simulink model "IEEE118_FULL_seed17_GFOL_RL_percgfor091_PyStable"  (R2023a)
(part 1 of 3)
settings: Solver=ode1  StartTime=0.0  StopTime=sim_config.Tsim  RelTol=1e-3
undefined symbols (not defined in the file): sim_config
libraries: myLibrary x561, spsThreePhaseVIMeasurementLib x250, spsPower3phInstantaneousLib x137, spspowerguiLib x1
settings Model: Creator=Francesca  LastModifiedBy=Francesca

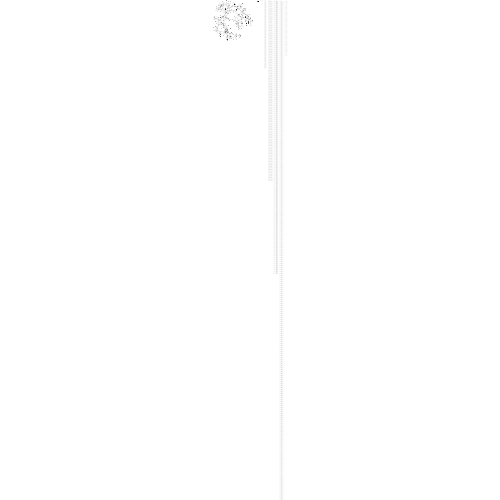
[thumbnail: Simulink's stored preview of the top-level diagram]
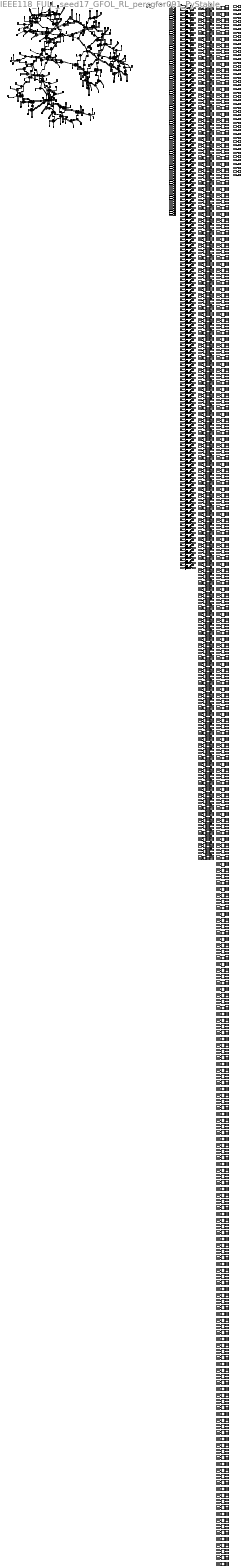
== system IEEE118_FULL_seed17_GFOL_RL_percgfor091_PyStable ==
  note: Line-to-Line Voltages
  note: Line-to-Neutral Voltages
  note: Power Measurements
  note: qd0 transforms
  note: omega
  BUS-1 : spsThreePhaseVIMeasurementLib/Three-Phase V-I Measurement  VoltageMeasurement=phase-to-phase  SetLabelV=on  LabelV=V_ll_1  Vpu=off  VpuLL=off  CurrentMeasurement=yes  SetLabelI=on  LabelI=I_1  Ipu=off  Pbase=100e6  Vbase=500e3  OutputType=Complex  PhasorSimulation=off  PSBequivalent=0
  BUS-100 : spsThreePhaseVIMeasurementLib/Three-Phase V-I Measurement  VoltageMeasurement=phase-to-phase  SetLabelV=on  LabelV=V_ll_100  Vpu=off  VpuLL=off  CurrentMeasurement=yes  SetLabelI=on  LabelI=I_100  Ipu=off  Pbase=100e6  Vbase=500e3  OutputType=Complex  PhasorSimulation=off  PSBequivalent=0
  BUS-101 : spsThreePhaseVIMeasurementLib/Three-Phase V-I Measurement  VoltageMeasurement=phase-to-phase  SetLabelV=on  LabelV=V_ll_101  Vpu=off  VpuLL=off  CurrentMeasurement=yes  SetLabelI=on  LabelI=I_101  Ipu=off  Pbase=100e6  Vbase=500e3  OutputType=Complex  PhasorSimulation=off  PSBequivalent=0
  BUS-102 : spsThreePhaseVIMeasurementLib/Three-Phase V-I Measurement  VoltageMeasurement=phase-to-phase  SetLabelV=on  LabelV=V_ll_102  Vpu=off  VpuLL=off  CurrentMeasurement=yes  SetLabelI=on  LabelI=I_102  Ipu=off  Pbase=100e6  Vbase=500e3  OutputType=Complex  PhasorSimulation=off  PSBequivalent=0
  BUS-103 : spsThreePhaseVIMeasurementLib/Three-Phase V-I Measurement  VoltageMeasurement=phase-to-phase  SetLabelV=on  LabelV=V_ll_103  Vpu=off  VpuLL=off  CurrentMeasurement=yes  SetLabelI=on  LabelI=I_103  Ipu=off  Pbase=100e6  Vbase=500e3  OutputType=Complex  PhasorSimulation=off  PSBequivalent=0
  BUS-104 : spsThreePhaseVIMeasurementLib/Three-Phase V-I Measurement  VoltageMeasurement=phase-to-phase  SetLabelV=on  LabelV=V_ll_104  Vpu=off  VpuLL=off  CurrentMeasurement=yes  SetLabelI=on  LabelI=I_104  Ipu=off  Pbase=100e6  Vbase=500e3  OutputType=Complex  PhasorSimulation=off  PSBequivalent=0
  BUS-105 : spsThreePhaseVIMeasurementLib/Three-Phase V-I Measurement  VoltageMeasurement=phase-to-phase  SetLabelV=on  LabelV=V_ll_105  Vpu=off  VpuLL=off  CurrentMeasurement=yes  SetLabelI=on  LabelI=I_105  Ipu=off  Pbase=100e6  Vbase=500e3  OutputType=Complex  PhasorSimulation=off  PSBequivalent=0
  BUS-106 : spsThreePhaseVIMeasurementLib/Three-Phase V-I Measurement  VoltageMeasurement=phase-to-phase  SetLabelV=on  LabelV=V_ll_106  Vpu=off  VpuLL=off  CurrentMeasurement=yes  SetLabelI=on  LabelI=I_106  Ipu=off  Pbase=100e6  Vbase=500e3  OutputType=Complex  PhasorSimulation=off  PSBequivalent=0
  BUS-107 : spsThreePhaseVIMeasurementLib/Three-Phase V-I Measurement  VoltageMeasurement=phase-to-phase  SetLabelV=on  LabelV=V_ll_107  Vpu=off  VpuLL=off  CurrentMeasurement=yes  SetLabelI=on  LabelI=I_107  Ipu=off  Pbase=100e6  Vbase=500e3  OutputType=Complex  PhasorSimulation=off  PSBequivalent=0
  BUS-108 : spsThreePhaseVIMeasurementLib/Three-Phase V-I Measurement  VoltageMeasurement=phase-to-phase  SetLabelV=on  LabelV=V_ll_108  Vpu=off  VpuLL=off  CurrentMeasurement=yes  SetLabelI=on  LabelI=I_108  Ipu=off  Pbase=100e6  Vbase=500e3  OutputType=Complex  PhasorSimulation=off  PSBequivalent=0
  BUS-109 : spsThreePhaseVIMeasurementLib/Three-Phase V-I Measurement  VoltageMeasurement=phase-to-phase  SetLabelV=on  LabelV=V_ll_109  Vpu=off  VpuLL=off  CurrentMeasurement=yes  SetLabelI=on  LabelI=I_109  Ipu=off  Pbase=100e6  Vbase=500e3  OutputType=Complex  PhasorSimulation=off  PSBequivalent=0
  BUS-11 : spsThreePhaseVIMeasurementLib/Three-Phase V-I Measurement  VoltageMeasurement=phase-to-phase  SetLabelV=on  LabelV=V_ll_11  Vpu=off  VpuLL=off  CurrentMeasurement=yes  SetLabelI=on  LabelI=I_11  Ipu=off  Pbase=100e6  Vbase=500e3  OutputType=Complex  PhasorSimulation=off  PSBequivalent=0
  BUS-110 : spsThreePhaseVIMeasurementLib/Three-Phase V-I Measurement  VoltageMeasurement=phase-to-phase  SetLabelV=on  LabelV=V_ll_110  Vpu=off  VpuLL=off  CurrentMeasurement=yes  SetLabelI=on  LabelI=I_110  Ipu=off  Pbase=100e6  Vbase=500e3  OutputType=Complex  PhasorSimulation=off  PSBequivalent=0
  BUS-112 : spsThreePhaseVIMeasurementLib/Three-Phase V-I Measurement  VoltageMeasurement=phase-to-phase  SetLabelV=on  LabelV=V_ll_112  Vpu=off  VpuLL=off  CurrentMeasurement=yes  SetLabelI=on  LabelI=I_112  Ipu=off  Pbase=100e6  Vbase=500e3  OutputType=Complex  PhasorSimulation=off  PSBequivalent=0
  BUS-113 : spsThreePhaseVIMeasurementLib/Three-Phase V-I Measurement  VoltageMeasurement=phase-to-phase  SetLabelV=on  LabelV=V_ll_113  Vpu=off  VpuLL=off  CurrentMeasurement=yes  SetLabelI=on  LabelI=I_113  Ipu=off  Pbase=100e6  Vbase=500e3  OutputType=Complex  PhasorSimulation=off  PSBequivalent=0
  BUS-114 : spsThreePhaseVIMeasurementLib/Three-Phase V-I Measurement  VoltageMeasurement=phase-to-phase  SetLabelV=on  LabelV=V_ll_114  Vpu=off  VpuLL=off  CurrentMeasurement=yes  SetLabelI=on  LabelI=I_114  Ipu=off  Pbase=100e6  Vbase=500e3  OutputType=Complex  PhasorSimulation=off  PSBequivalent=0
  BUS-115 : spsThreePhaseVIMeasurementLib/Three-Phase V-I Measurement  VoltageMeasurement=phase-to-phase  SetLabelV=on  LabelV=V_ll_115  Vpu=off  VpuLL=off  CurrentMeasurement=yes  SetLabelI=on  LabelI=I_115  Ipu=off  Pbase=100e6  Vbase=500e3  OutputType=Complex  PhasorSimulation=off  PSBequivalent=0
  BUS-117 : spsThreePhaseVIMeasurementLib/Three-Phase V-I Measurement  VoltageMeasurement=phase-to-phase  SetLabelV=on  LabelV=V_ll_117  Vpu=off  VpuLL=off  CurrentMeasurement=yes  SetLabelI=on  LabelI=I_117  Ipu=off  Pbase=100e6  Vbase=500e3  OutputType=Complex  PhasorSimulation=off  PSBequivalent=0
  BUS-118 : spsThreePhaseVIMeasurementLib/Three-Phase V-I Measurement  VoltageMeasurement=phase-to-phase  SetLabelV=on  LabelV=V_ll_118  Vpu=off  VpuLL=off  CurrentMeasurement=yes  SetLabelI=on  LabelI=I_118  Ipu=off  Pbase=100e6  Vbase=500e3  OutputType=Complex  PhasorSimulation=off  PSBequivalent=0
  BUS-12 : spsThreePhaseVIMeasurementLib/Three-Phase V-I Measurement  VoltageMeasurement=phase-to-phase  SetLabelV=on  LabelV=V_ll_12  Vpu=off  VpuLL=off  CurrentMeasurement=yes  SetLabelI=on  LabelI=I_12  Ipu=off  Pbase=100e6  Vbase=500e3  OutputType=Complex  PhasorSimulation=off  PSBequivalent=0
  BUS-13 : spsThreePhaseVIMeasurementLib/Three-Phase V-I Measurement  VoltageMeasurement=phase-to-phase  SetLabelV=on  LabelV=V_ll_13  Vpu=off  VpuLL=off  CurrentMeasurement=yes  SetLabelI=on  LabelI=I_13  Ipu=off  Pbase=100e6  Vbase=500e3  OutputType=Complex  PhasorSimulation=off  PSBequivalent=0
  BUS-14 : spsThreePhaseVIMeasurementLib/Three-Phase V-I Measurement  VoltageMeasurement=phase-to-phase  SetLabelV=on  LabelV=V_ll_14  Vpu=off  VpuLL=off  CurrentMeasurement=yes  SetLabelI=on  LabelI=I_14  Ipu=off  Pbase=100e6  Vbase=500e3  OutputType=Complex  PhasorSimulation=off  PSBequivalent=0
  BUS-15 : spsThreePhaseVIMeasurementLib/Three-Phase V-I Measurement  VoltageMeasurement=phase-to-phase  SetLabelV=on  LabelV=V_ll_15  Vpu=off  VpuLL=off  CurrentMeasurement=yes  SetLabelI=on  LabelI=I_15  Ipu=off  Pbase=100e6  Vbase=500e3  OutputType=Complex  PhasorSimulation=off  PSBequivalent=0
  BUS-16 : spsThreePhaseVIMeasurementLib/Three-Phase V-I Measurement  VoltageMeasurement=phase-to-phase  SetLabelV=on  LabelV=V_ll_16  Vpu=off  VpuLL=off  CurrentMeasurement=yes  SetLabelI=on  LabelI=I_16  Ipu=off  Pbase=100e6  Vbase=500e3  OutputType=Complex  PhasorSimulation=off  PSBequivalent=0
  BUS-17 : spsThreePhaseVIMeasurementLib/Three-Phase V-I Measurement  VoltageMeasurement=phase-to-phase  SetLabelV=on  LabelV=V_ll_17  Vpu=off  VpuLL=off  CurrentMeasurement=yes  SetLabelI=on  LabelI=I_17  Ipu=off  Pbase=100e6  Vbase=500e3  OutputType=Complex  PhasorSimulation=off  PSBequivalent=0
  BUS-18 : spsThreePhaseVIMeasurementLib/Three-Phase V-I Measurement  VoltageMeasurement=phase-to-phase  SetLabelV=on  LabelV=V_ll_18  Vpu=off  VpuLL=off  CurrentMeasurement=yes  SetLabelI=on  LabelI=I_18  Ipu=off  Pbase=100e6  Vbase=500e3  OutputType=Complex  PhasorSimulation=off  PSBequivalent=0
  BUS-19 : spsThreePhaseVIMeasurementLib/Three-Phase V-I Measurement  VoltageMeasurement=phase-to-phase  SetLabelV=on  LabelV=V_ll_19  Vpu=off  VpuLL=off  CurrentMeasurement=yes  SetLabelI=on  LabelI=I_19  Ipu=off  Pbase=100e6  Vbase=500e3  OutputType=Complex  PhasorSimulation=off  PSBequivalent=0
  BUS-2 : spsThreePhaseVIMeasurementLib/Three-Phase V-I Measurement  VoltageMeasurement=phase-to-phase  SetLabelV=on  LabelV=V_ll_2  Vpu=off  VpuLL=off  CurrentMeasurement=yes  SetLabelI=on  LabelI=I_2  Ipu=off  Pbase=100e6  Vbase=500e3  OutputType=Complex  PhasorSimulation=off  PSBequivalent=0
  BUS-20 : spsThreePhaseVIMeasurementLib/Three-Phase V-I Measurement  VoltageMeasurement=phase-to-phase  SetLabelV=on  LabelV=V_ll_20  Vpu=off  VpuLL=off  CurrentMeasurement=yes  SetLabelI=on  LabelI=I_20  Ipu=off  Pbase=100e6  Vbase=500e3  OutputType=Complex  PhasorSimulation=off  PSBequivalent=0
  BUS-21 : spsThreePhaseVIMeasurementLib/Three-Phase V-I Measurement  VoltageMeasurement=phase-to-phase  SetLabelV=on  LabelV=V_ll_21  Vpu=off  VpuLL=off  CurrentMeasurement=yes  SetLabelI=on  LabelI=I_21  Ipu=off  Pbase=100e6  Vbase=500e3  OutputType=Complex  PhasorSimulation=off  PSBequivalent=0
  BUS-22 : spsThreePhaseVIMeasurementLib/Three-Phase V-I Measurement  VoltageMeasurement=phase-to-phase  SetLabelV=on  LabelV=V_ll_22  Vpu=off  VpuLL=off  CurrentMeasurement=yes  SetLabelI=on  LabelI=I_22  Ipu=off  Pbase=100e6  Vbase=500e3  OutputType=Complex  PhasorSimulation=off  PSBequivalent=0
  BUS-23 : spsThreePhaseVIMeasurementLib/Three-Phase V-I Measurement  VoltageMeasurement=phase-to-phase  SetLabelV=on  LabelV=V_ll_23  Vpu=off  VpuLL=off  CurrentMeasurement=yes  SetLabelI=on  LabelI=I_23  Ipu=off  Pbase=100e6  Vbase=500e3  OutputType=Complex  PhasorSimulation=off  PSBequivalent=0
  BUS-24 : spsThreePhaseVIMeasurementLib/Three-Phase V-I Measurement  VoltageMeasurement=phase-to-phase  SetLabelV=on  LabelV=V_ll_24  Vpu=off  VpuLL=off  CurrentMeasurement=yes  SetLabelI=on  LabelI=I_24  Ipu=off  Pbase=100e6  Vbase=500e3  OutputType=Complex  PhasorSimulation=off  PSBequivalent=0
  BUS-25 : spsThreePhaseVIMeasurementLib/Three-Phase V-I Measurement  VoltageMeasurement=phase-to-phase  SetLabelV=on  LabelV=V_ll_25  Vpu=off  VpuLL=off  CurrentMeasurement=yes  SetLabelI=on  LabelI=I_25  Ipu=off  Pbase=100e6  Vbase=500e3  OutputType=Complex  PhasorSimulation=off  PSBequivalent=0
  BUS-26 : spsThreePhaseVIMeasurementLib/Three-Phase V-I Measurement  VoltageMeasurement=phase-to-phase  SetLabelV=on  LabelV=V_ll_26  Vpu=off  VpuLL=off  CurrentMeasurement=yes  SetLabelI=on  LabelI=I_26  Ipu=off  Pbase=100e6  Vbase=500e3  OutputType=Complex  PhasorSimulation=off  PSBequivalent=0
  BUS-27 : spsThreePhaseVIMeasurementLib/Three-Phase V-I Measurement  VoltageMeasurement=phase-to-phase  SetLabelV=on  LabelV=V_ll_27  Vpu=off  VpuLL=off  CurrentMeasurement=yes  SetLabelI=on  LabelI=I_27  Ipu=off  Pbase=100e6  Vbase=500e3  OutputType=Complex  PhasorSimulation=off  PSBequivalent=0
  BUS-28 : spsThreePhaseVIMeasurementLib/Three-Phase V-I Measurement  VoltageMeasurement=phase-to-phase  SetLabelV=on  LabelV=V_ll_28  Vpu=off  VpuLL=off  CurrentMeasurement=yes  SetLabelI=on  LabelI=I_28  Ipu=off  Pbase=100e6  Vbase=500e3  OutputType=Complex  PhasorSimulation=off  PSBequivalent=0
  BUS-29 : spsThreePhaseVIMeasurementLib/Three-Phase V-I Measurement  VoltageMeasurement=phase-to-phase  SetLabelV=on  LabelV=V_ll_29  Vpu=off  VpuLL=off  CurrentMeasurement=yes  SetLabelI=on  LabelI=I_29  Ipu=off  Pbase=100e6  Vbase=500e3  OutputType=Complex  PhasorSimulation=off  PSBequivalent=0
  BUS-3 : spsThreePhaseVIMeasurementLib/Three-Phase V-I Measurement  VoltageMeasurement=phase-to-phase  SetLabelV=on  LabelV=V_ll_3  Vpu=off  VpuLL=off  CurrentMeasurement=yes  SetLabelI=on  LabelI=I_3  Ipu=off  Pbase=100e6  Vbase=500e3  OutputType=Complex  PhasorSimulation=off  PSBequivalent=0
  BUS-30 : spsThreePhaseVIMeasurementLib/Three-Phase V-I Measurement  VoltageMeasurement=phase-to-phase  SetLabelV=on  LabelV=V_ll_30  Vpu=off  VpuLL=off  CurrentMeasurement=yes  SetLabelI=on  LabelI=I_30  Ipu=off  Pbase=100e6  Vbase=500e3  OutputType=Complex  PhasorSimulation=off  PSBequivalent=0
  BUS-31 : spsThreePhaseVIMeasurementLib/Three-Phase V-I Measurement  VoltageMeasurement=phase-to-phase  SetLabelV=on  LabelV=V_ll_31  Vpu=off  VpuLL=off  CurrentMeasurement=yes  SetLabelI=on  LabelI=I_31  Ipu=off  Pbase=100e6  Vbase=500e3  OutputType=Complex  PhasorSimulation=off  PSBequivalent=0
  BUS-32 : spsThreePhaseVIMeasurementLib/Three-Phase V-I Measurement  VoltageMeasurement=phase-to-phase  SetLabelV=on  LabelV=V_ll_32  Vpu=off  VpuLL=off  CurrentMeasurement=yes  SetLabelI=on  LabelI=I_32  Ipu=off  Pbase=100e6  Vbase=500e3  OutputType=Complex  PhasorSimulation=off  PSBequivalent=0
  BUS-33 : spsThreePhaseVIMeasurementLib/Three-Phase V-I Measurement  VoltageMeasurement=phase-to-phase  SetLabelV=on  LabelV=V_ll_33  Vpu=off  VpuLL=off  CurrentMeasurement=yes  SetLabelI=on  LabelI=I_33  Ipu=off  Pbase=100e6  Vbase=500e3  OutputType=Complex  PhasorSimulation=off  PSBequivalent=0
  BUS-34 : spsThreePhaseVIMeasurementLib/Three-Phase V-I Measurement  VoltageMeasurement=phase-to-phase  SetLabelV=on  LabelV=V_ll_34  Vpu=off  VpuLL=off  CurrentMeasurement=yes  SetLabelI=on  LabelI=I_34  Ipu=off  Pbase=100e6  Vbase=500e3  OutputType=Complex  PhasorSimulation=off  PSBequivalent=0
  BUS-35 : spsThreePhaseVIMeasurementLib/Three-Phase V-I Measurement  VoltageMeasurement=phase-to-phase  SetLabelV=on  LabelV=V_ll_35  Vpu=off  VpuLL=off  CurrentMeasurement=yes  SetLabelI=on  LabelI=I_35  Ipu=off  Pbase=100e6  Vbase=500e3  OutputType=Complex  PhasorSimulation=off  PSBequivalent=0
  BUS-36 : spsThreePhaseVIMeasurementLib/Three-Phase V-I Measurement  VoltageMeasurement=phase-to-phase  SetLabelV=on  LabelV=V_ll_36  Vpu=off  VpuLL=off  CurrentMeasurement=yes  SetLabelI=on  LabelI=I_36  Ipu=off  Pbase=100e6  Vbase=500e3  OutputType=Complex  PhasorSimulation=off  PSBequivalent=0
  BUS-37 : spsThreePhaseVIMeasurementLib/Three-Phase V-I Measurement  VoltageMeasurement=phase-to-phase  SetLabelV=on  LabelV=V_ll_37  Vpu=off  VpuLL=off  CurrentMeasurement=yes  SetLabelI=on  LabelI=I_37  Ipu=off  Pbase=100e6  Vbase=500e3  OutputType=Complex  PhasorSimulation=off  PSBequivalent=0
  BUS-38 : spsThreePhaseVIMeasurementLib/Three-Phase V-I Measurement  VoltageMeasurement=phase-to-phase  SetLabelV=on  LabelV=V_ll_38  Vpu=off  VpuLL=off  CurrentMeasurement=yes  SetLabelI=on  LabelI=I_38  Ipu=off  Pbase=100e6  Vbase=500e3  OutputType=Complex  PhasorSimulation=off  PSBequivalent=0
  BUS-39 : spsThreePhaseVIMeasurementLib/Three-Phase V-I Measurement  VoltageMeasurement=phase-to-phase  SetLabelV=on  LabelV=V_ll_39  Vpu=off  VpuLL=off  CurrentMeasurement=yes  SetLabelI=on  LabelI=I_39  Ipu=off  Pbase=100e6  Vbase=500e3  OutputType=Complex  PhasorSimulation=off  PSBequivalent=0
  BUS-4 : spsThreePhaseVIMeasurementLib/Three-Phase V-I Measurement  VoltageMeasurement=phase-to-phase  SetLabelV=on  LabelV=V_ll_4  Vpu=off  VpuLL=off  CurrentMeasurement=yes  SetLabelI=on  LabelI=I_4  Ipu=off  Pbase=100e6  Vbase=500e3  OutputType=Complex  PhasorSimulation=off  PSBequivalent=0
  BUS-40 : spsThreePhaseVIMeasurementLib/Three-Phase V-I Measurement  VoltageMeasurement=phase-to-phase  SetLabelV=on  LabelV=V_ll_40  Vpu=off  VpuLL=off  CurrentMeasurement=yes  SetLabelI=on  LabelI=I_40  Ipu=off  Pbase=100e6  Vbase=500e3  OutputType=Complex  PhasorSimulation=off  PSBequivalent=0
  BUS-41 : spsThreePhaseVIMeasurementLib/Three-Phase V-I Measurement  VoltageMeasurement=phase-to-phase  SetLabelV=on  LabelV=V_ll_41  Vpu=off  VpuLL=off  CurrentMeasurement=yes  SetLabelI=on  LabelI=I_41  Ipu=off  Pbase=100e6  Vbase=500e3  OutputType=Complex  PhasorSimulation=off  PSBequivalent=0
  BUS-42 : spsThreePhaseVIMeasurementLib/Three-Phase V-I Measurement  VoltageMeasurement=phase-to-phase  SetLabelV=on  LabelV=V_ll_42  Vpu=off  VpuLL=off  CurrentMeasurement=yes  SetLabelI=on  LabelI=I_42  Ipu=off  Pbase=100e6  Vbase=500e3  OutputType=Complex  PhasorSimulation=off  PSBequivalent=0
  BUS-43 : spsThreePhaseVIMeasurementLib/Three-Phase V-I Measurement  VoltageMeasurement=phase-to-phase  SetLabelV=on  LabelV=V_ll_43  Vpu=off  VpuLL=off  CurrentMeasurement=yes  SetLabelI=on  LabelI=I_43  Ipu=off  Pbase=100e6  Vbase=500e3  OutputType=Complex  PhasorSimulation=off  PSBequivalent=0
  BUS-44 : spsThreePhaseVIMeasurementLib/Three-Phase V-I Measurement  VoltageMeasurement=phase-to-phase  SetLabelV=on  LabelV=V_ll_44  Vpu=off  VpuLL=off  CurrentMeasurement=yes  SetLabelI=on  LabelI=I_44  Ipu=off  Pbase=100e6  Vbase=500e3  OutputType=Complex  PhasorSimulation=off  PSBequivalent=0
  BUS-45 : spsThreePhaseVIMeasurementLib/Three-Phase V-I Measurement  VoltageMeasurement=phase-to-phase  SetLabelV=on  LabelV=V_ll_45  Vpu=off  VpuLL=off  CurrentMeasurement=yes  SetLabelI=on  LabelI=I_45  Ipu=off  Pbase=100e6  Vbase=500e3  OutputType=Complex  PhasorSimulation=off  PSBequivalent=0
  BUS-46 : spsThreePhaseVIMeasurementLib/Three-Phase V-I Measurement  VoltageMeasurement=phase-to-phase  SetLabelV=on  LabelV=V_ll_46  Vpu=off  VpuLL=off  CurrentMeasurement=yes  SetLabelI=on  LabelI=I_46  Ipu=off  Pbase=100e6  Vbase=500e3  OutputType=Complex  PhasorSimulation=off  PSBequivalent=0
  BUS-47 : spsThreePhaseVIMeasurementLib/Three-Phase V-I Measurement  VoltageMeasurement=phase-to-phase  SetLabelV=on  LabelV=V_ll_47  Vpu=off  VpuLL=off  CurrentMeasurement=yes  SetLabelI=on  LabelI=I_47  Ipu=off  Pbase=100e6  Vbase=500e3  OutputType=Complex  PhasorSimulation=off  PSBequivalent=0
  BUS-48 : spsThreePhaseVIMeasurementLib/Three-Phase V-I Measurement  VoltageMeasurement=phase-to-phase  SetLabelV=on  LabelV=V_ll_48  Vpu=off  VpuLL=off  CurrentMeasurement=yes  SetLabelI=on  LabelI=I_48  Ipu=off  Pbase=100e6  Vbase=500e3  OutputType=Complex  PhasorSimulation=off  PSBequivalent=0
  BUS-49 : spsThreePhaseVIMeasurementLib/Three-Phase V-I Measurement  VoltageMeasurement=phase-to-phase  SetLabelV=on  LabelV=V_ll_49  Vpu=off  VpuLL=off  CurrentMeasurement=yes  SetLabelI=on  LabelI=I_49  Ipu=off  Pbase=100e6  Vbase=500e3  OutputType=Complex  PhasorSimulation=off  PSBequivalent=0
  BUS-5 : spsThreePhaseVIMeasurementLib/Three-Phase V-I Measurement  VoltageMeasurement=phase-to-phase  SetLabelV=on  LabelV=V_ll_5  Vpu=off  VpuLL=off  CurrentMeasurement=yes  SetLabelI=on  LabelI=I_5  Ipu=off  Pbase=100e6  Vbase=500e3  OutputType=Complex  PhasorSimulation=off  PSBequivalent=0
  BUS-50 : spsThreePhaseVIMeasurementLib/Three-Phase V-I Measurement  VoltageMeasurement=phase-to-phase  SetLabelV=on  LabelV=V_ll_50  Vpu=off  VpuLL=off  CurrentMeasurement=yes  SetLabelI=on  LabelI=I_50  Ipu=off  Pbase=100e6  Vbase=500e3  OutputType=Complex  PhasorSimulation=off  PSBequivalent=0
  BUS-51 : spsThreePhaseVIMeasurementLib/Three-Phase V-I Measurement  VoltageMeasurement=phase-to-phase  SetLabelV=on  LabelV=V_ll_51  Vpu=off  VpuLL=off  CurrentMeasurement=yes  SetLabelI=on  LabelI=I_51  Ipu=off  Pbase=100e6  Vbase=500e3  OutputType=Complex  PhasorSimulation=off  PSBequivalent=0
  BUS-52 : spsThreePhaseVIMeasurementLib/Three-Phase V-I Measurement  VoltageMeasurement=phase-to-phase  SetLabelV=on  LabelV=V_ll_52  Vpu=off  VpuLL=off  CurrentMeasurement=yes  SetLabelI=on  LabelI=I_52  Ipu=off  Pbase=100e6  Vbase=500e3  OutputType=Complex  PhasorSimulation=off  PSBequivalent=0
  BUS-53 : spsThreePhaseVIMeasurementLib/Three-Phase V-I Measurement  VoltageMeasurement=phase-to-phase  SetLabelV=on  LabelV=V_ll_53  Vpu=off  VpuLL=off  CurrentMeasurement=yes  SetLabelI=on  LabelI=I_53  Ipu=off  Pbase=100e6  Vbase=500e3  OutputType=Complex  PhasorSimulation=off  PSBequivalent=0
  BUS-54 : spsThreePhaseVIMeasurementLib/Three-Phase V-I Measurement  VoltageMeasurement=phase-to-phase  SetLabelV=on  LabelV=V_ll_54  Vpu=off  VpuLL=off  CurrentMeasurement=yes  SetLabelI=on  LabelI=I_54  Ipu=off  Pbase=100e6  Vbase=500e3  OutputType=Complex  PhasorSimulation=off  PSBequivalent=0
  BUS-55 : spsThreePhaseVIMeasurementLib/Three-Phase V-I Measurement  VoltageMeasurement=phase-to-phase  SetLabelV=on  LabelV=V_ll_55  Vpu=off  VpuLL=off  CurrentMeasurement=yes  SetLabelI=on  LabelI=I_55  Ipu=off  Pbase=100e6  Vbase=500e3  OutputType=Complex  PhasorSimulation=off  PSBequivalent=0
  BUS-56 : spsThreePhaseVIMeasurementLib/Three-Phase V-I Measurement  VoltageMeasurement=phase-to-phase  SetLabelV=on  LabelV=V_ll_56  Vpu=off  VpuLL=off  CurrentMeasurement=yes  SetLabelI=on  LabelI=I_56  Ipu=off  Pbase=100e6  Vbase=500e3  OutputType=Complex  PhasorSimulation=off  PSBequivalent=0
  BUS-57 : spsThreePhaseVIMeasurementLib/Three-Phase V-I Measurement  VoltageMeasurement=phase-to-phase  SetLabelV=on  LabelV=V_ll_57  Vpu=off  VpuLL=off  CurrentMeasurement=yes  SetLabelI=on  LabelI=I_57  Ipu=off  Pbase=100e6  Vbase=500e3  OutputType=Complex  PhasorSimulation=off  PSBequivalent=0
  BUS-58 : spsThreePhaseVIMeasurementLib/Three-Phase V-I Measurement  VoltageMeasurement=phase-to-phase  SetLabelV=on  LabelV=V_ll_58  Vpu=off  VpuLL=off  CurrentMeasurement=yes  SetLabelI=on  LabelI=I_58  Ipu=off  Pbase=100e6  Vbase=500e3  OutputType=Complex  PhasorSimulation=off  PSBequivalent=0
  BUS-59 : spsThreePhaseVIMeasurementLib/Three-Phase V-I Measurement  VoltageMeasurement=phase-to-phase  SetLabelV=on  LabelV=V_ll_59  Vpu=off  VpuLL=off  CurrentMeasurement=yes  SetLabelI=on  LabelI=I_59  Ipu=off  Pbase=100e6  Vbase=500e3  OutputType=Complex  PhasorSimulation=off  PSBequivalent=0
  BUS-6 : spsThreePhaseVIMeasurementLib/Three-Phase V-I Measurement  VoltageMeasurement=phase-to-phase  SetLabelV=on  LabelV=V_ll_6  Vpu=off  VpuLL=off  CurrentMeasurement=yes  SetLabelI=on  LabelI=I_6  Ipu=off  Pbase=100e6  Vbase=500e3  OutputType=Complex  PhasorSimulation=off  PSBequivalent=0
  BUS-60 : spsThreePhaseVIMeasurementLib/Three-Phase V-I Measurement  VoltageMeasurement=phase-to-phase  SetLabelV=on  LabelV=V_ll_60  Vpu=off  VpuLL=off  CurrentMeasurement=yes  SetLabelI=on  LabelI=I_60  Ipu=off  Pbase=100e6  Vbase=500e3  OutputType=Complex  PhasorSimulation=off  PSBequivalent=0
  BUS-61 : spsThreePhaseVIMeasurementLib/Three-Phase V-I Measurement  VoltageMeasurement=phase-to-phase  SetLabelV=on  LabelV=V_ll_61  Vpu=off  VpuLL=off  CurrentMeasurement=yes  SetLabelI=on  LabelI=I_61  Ipu=off  Pbase=100e6  Vbase=500e3  OutputType=Complex  PhasorSimulation=off  PSBequivalent=0
  BUS-62 : spsThreePhaseVIMeasurementLib/Three-Phase V-I Measurement  VoltageMeasurement=phase-to-phase  SetLabelV=on  LabelV=V_ll_62  Vpu=off  VpuLL=off  CurrentMeasurement=yes  SetLabelI=on  LabelI=I_62  Ipu=off  Pbase=100e6  Vbase=500e3  OutputType=Complex  PhasorSimulation=off  PSBequivalent=0
  BUS-63 : spsThreePhaseVIMeasurementLib/Three-Phase V-I Measurement  VoltageMeasurement=phase-to-phase  SetLabelV=on  LabelV=V_ll_63  Vpu=off  VpuLL=off  CurrentMeasurement=yes  SetLabelI=on  LabelI=I_63  Ipu=off  Pbase=100e6  Vbase=500e3  OutputType=Complex  PhasorSimulation=off  PSBequivalent=0
  BUS-64 : spsThreePhaseVIMeasurementLib/Three-Phase V-I Measurement  VoltageMeasurement=phase-to-phase  SetLabelV=on  LabelV=V_ll_64  Vpu=off  VpuLL=off  CurrentMeasurement=yes  SetLabelI=on  LabelI=I_64  Ipu=off  Pbase=100e6  Vbase=500e3  OutputType=Complex  PhasorSimulation=off  PSBequivalent=0
  BUS-65 : spsThreePhaseVIMeasurementLib/Three-Phase V-I Measurement  VoltageMeasurement=phase-to-phase  SetLabelV=on  LabelV=V_ll_65  Vpu=off  VpuLL=off  CurrentMeasurement=yes  SetLabelI=on  LabelI=I_65  Ipu=off  Pbase=100e6  Vbase=500e3  OutputType=Complex  PhasorSimulation=off  PSBequivalent=0
  BUS-66 : spsThreePhaseVIMeasurementLib/Three-Phase V-I Measurement  VoltageMeasurement=phase-to-phase  SetLabelV=on  LabelV=V_ll_66  Vpu=off  VpuLL=off  CurrentMeasurement=yes  SetLabelI=on  LabelI=I_66  Ipu=off  Pbase=100e6  Vbase=500e3  OutputType=Complex  PhasorSimulation=off  PSBequivalent=0
  BUS-67 : spsThreePhaseVIMeasurementLib/Three-Phase V-I Measurement  VoltageMeasurement=phase-to-phase  SetLabelV=on  LabelV=V_ll_67  Vpu=off  VpuLL=off  CurrentMeasurement=yes  SetLabelI=on  LabelI=I_67  Ipu=off  Pbase=100e6  Vbase=500e3  OutputType=Complex  PhasorSimulation=off  PSBequivalent=0
  BUS-68 : spsThreePhaseVIMeasurementLib/Three-Phase V-I Measurement  VoltageMeasurement=phase-to-phase  SetLabelV=on  LabelV=V_ll_68  Vpu=off  VpuLL=off  CurrentMeasurement=yes  SetLabelI=on  LabelI=I_68  Ipu=off  Pbase=100e6  Vbase=500e3  OutputType=Complex  PhasorSimulation=off  PSBequivalent=0
  BUS-69 : spsThreePhaseVIMeasurementLib/Three-Phase V-I Measurement  VoltageMeasurement=phase-to-phase  SetLabelV=on  LabelV=V_ll_69  Vpu=off  VpuLL=off  CurrentMeasurement=yes  SetLabelI=on  LabelI=I_69  Ipu=off  Pbase=100e6  Vbase=500e3  OutputType=Complex  PhasorSimulation=off  PSBequivalent=0
  BUS-7 : spsThreePhaseVIMeasurementLib/Three-Phase V-I Measurement  VoltageMeasurement=phase-to-phase  SetLabelV=on  LabelV=V_ll_7  Vpu=off  VpuLL=off  CurrentMeasurement=yes  SetLabelI=on  LabelI=I_7  Ipu=off  Pbase=100e6  Vbase=500e3  OutputType=Complex  PhasorSimulation=off  PSBequivalent=0
  BUS-70 : spsThreePhaseVIMeasurementLib/Three-Phase V-I Measurement  VoltageMeasurement=phase-to-phase  SetLabelV=on  LabelV=V_ll_70  Vpu=off  VpuLL=off  CurrentMeasurement=yes  SetLabelI=on  LabelI=I_70  Ipu=off  Pbase=100e6  Vbase=500e3  OutputType=Complex  PhasorSimulation=off  PSBequivalent=0
  BUS-71 : spsThreePhaseVIMeasurementLib/Three-Phase V-I Measurement  VoltageMeasurement=phase-to-phase  SetLabelV=on  LabelV=V_ll_71  Vpu=off  VpuLL=off  CurrentMeasurement=yes  SetLabelI=on  LabelI=I_71  Ipu=off  Pbase=100e6  Vbase=500e3  OutputType=Complex  PhasorSimulation=off  PSBequivalent=0
  BUS-72 : spsThreePhaseVIMeasurementLib/Three-Phase V-I Measurement  VoltageMeasurement=phase-to-phase  SetLabelV=on  LabelV=V_ll_72  Vpu=off  VpuLL=off  CurrentMeasurement=yes  SetLabelI=on  LabelI=I_72  Ipu=off  Pbase=100e6  Vbase=500e3  OutputType=Complex  PhasorSimulation=off  PSBequivalent=0
  BUS-73 : spsThreePhaseVIMeasurementLib/Three-Phase V-I Measurement  VoltageMeasurement=phase-to-phase  SetLabelV=on  LabelV=V_ll_73  Vpu=off  VpuLL=off  CurrentMeasurement=yes  SetLabelI=on  LabelI=I_73  Ipu=off  Pbase=100e6  Vbase=500e3  OutputType=Complex  PhasorSimulation=off  PSBequivalent=0
  BUS-74 : spsThreePhaseVIMeasurementLib/Three-Phase V-I Measurement  VoltageMeasurement=phase-to-phase  SetLabelV=on  LabelV=V_ll_74  Vpu=off  VpuLL=off  CurrentMeasurement=yes  SetLabelI=on  LabelI=I_74  Ipu=off  Pbase=100e6  Vbase=500e3  OutputType=Complex  PhasorSimulation=off  PSBequivalent=0
  BUS-75 : spsThreePhaseVIMeasurementLib/Three-Phase V-I Measurement  VoltageMeasurement=phase-to-phase  SetLabelV=on  LabelV=V_ll_75  Vpu=off  VpuLL=off  CurrentMeasurement=yes  SetLabelI=on  LabelI=I_75  Ipu=off  Pbase=100e6  Vbase=500e3  OutputType=Complex  PhasorSimulation=off  PSBequivalent=0
  BUS-76 : spsThreePhaseVIMeasurementLib/Three-Phase V-I Measurement  VoltageMeasurement=phase-to-phase  SetLabelV=on  LabelV=V_ll_76  Vpu=off  VpuLL=off  CurrentMeasurement=yes  SetLabelI=on  LabelI=I_76  Ipu=off  Pbase=100e6  Vbase=500e3  OutputType=Complex  PhasorSimulation=off  PSBequivalent=0
  BUS-77 : spsThreePhaseVIMeasurementLib/Three-Phase V-I Measurement  VoltageMeasurement=phase-to-phase  SetLabelV=on  LabelV=V_ll_77  Vpu=off  VpuLL=off  CurrentMeasurement=yes  SetLabelI=on  LabelI=I_77  Ipu=off  Pbase=100e6  Vbase=500e3  OutputType=Complex  PhasorSimulation=off  PSBequivalent=0
  BUS-78 : spsThreePhaseVIMeasurementLib/Three-Phase V-I Measurement  VoltageMeasurement=phase-to-phase  SetLabelV=on  LabelV=V_ll_78  Vpu=off  VpuLL=off  CurrentMeasurement=yes  SetLabelI=on  LabelI=I_78  Ipu=off  Pbase=100e6  Vbase=500e3  OutputType=Complex  PhasorSimulation=off  PSBequivalent=0
  BUS-79 : spsThreePhaseVIMeasurementLib/Three-Phase V-I Measurement  VoltageMeasurement=phase-to-phase  SetLabelV=on  LabelV=V_ll_79  Vpu=off  VpuLL=off  CurrentMeasurement=yes  SetLabelI=on  LabelI=I_79  Ipu=off  Pbase=100e6  Vbase=500e3  OutputType=Complex  PhasorSimulation=off  PSBequivalent=0
  BUS-8 : spsThreePhaseVIMeasurementLib/Three-Phase V-I Measurement  VoltageMeasurement=phase-to-phase  SetLabelV=on  LabelV=V_ll_8  Vpu=off  VpuLL=off  CurrentMeasurement=yes  SetLabelI=on  LabelI=I_8  Ipu=off  Pbase=100e6  Vbase=500e3  OutputType=Complex  PhasorSimulation=off  PSBequivalent=0
  BUS-80 : spsThreePhaseVIMeasurementLib/Three-Phase V-I Measurement  VoltageMeasurement=phase-to-phase  SetLabelV=on  LabelV=V_ll_80  Vpu=off  VpuLL=off  CurrentMeasurement=yes  SetLabelI=on  LabelI=I_80  Ipu=off  Pbase=100e6  Vbase=500e3  OutputType=Complex  PhasorSimulation=off  PSBequivalent=0
  BUS-81 : spsThreePhaseVIMeasurementLib/Three-Phase V-I Measurement  VoltageMeasurement=phase-to-phase  SetLabelV=on  LabelV=V_ll_81  Vpu=off  VpuLL=off  CurrentMeasurement=yes  SetLabelI=on  LabelI=I_81  Ipu=off  Pbase=100e6  Vbase=500e3  OutputType=Complex  PhasorSimulation=off  PSBequivalent=0
  BUS-82 : spsThreePhaseVIMeasurementLib/Three-Phase V-I Measurement  VoltageMeasurement=phase-to-phase  SetLabelV=on  LabelV=V_ll_82  Vpu=off  VpuLL=off  CurrentMeasurement=yes  SetLabelI=on  LabelI=I_82  Ipu=off  Pbase=100e6  Vbase=500e3  OutputType=Complex  PhasorSimulation=off  PSBequivalent=0
  BUS-83 : spsThreePhaseVIMeasurementLib/Three-Phase V-I Measurement  VoltageMeasurement=phase-to-phase  SetLabelV=on  LabelV=V_ll_83  Vpu=off  VpuLL=off  CurrentMeasurement=yes  SetLabelI=on  LabelI=I_83  Ipu=off  Pbase=100e6  Vbase=500e3  OutputType=Complex  PhasorSimulation=off  PSBequivalent=0
  BUS-84 : spsThreePhaseVIMeasurementLib/Three-Phase V-I Measurement  VoltageMeasurement=phase-to-phase  SetLabelV=on  LabelV=V_ll_84  Vpu=off  VpuLL=off  CurrentMeasurement=yes  SetLabelI=on  LabelI=I_84  Ipu=off  Pbase=100e6  Vbase=500e3  OutputType=Complex  PhasorSimulation=off  PSBequivalent=0
  BUS-85 : spsThreePhaseVIMeasurementLib/Three-Phase V-I Measurement  VoltageMeasurement=phase-to-phase  SetLabelV=on  LabelV=V_ll_85  Vpu=off  VpuLL=off  CurrentMeasurement=yes  SetLabelI=on  LabelI=I_85  Ipu=off  Pbase=100e6  Vbase=500e3  OutputType=Complex  PhasorSimulation=off  PSBequivalent=0
  BUS-86 : spsThreePhaseVIMeasurementLib/Three-Phase V-I Measurement  VoltageMeasurement=phase-to-phase  SetLabelV=on  LabelV=V_ll_86  Vpu=off  VpuLL=off  CurrentMeasurement=yes  SetLabelI=on  LabelI=I_86  Ipu=off  Pbase=100e6  Vbase=500e3  OutputType=Complex  PhasorSimulation=off  PSBequivalent=0
  BUS-88 : spsThreePhaseVIMeasurementLib/Three-Phase V-I Measurement  VoltageMeasurement=phase-to-phase  SetLabelV=on  LabelV=V_ll_88  Vpu=off  VpuLL=off  CurrentMeasurement=yes  SetLabelI=on  LabelI=I_88  Ipu=off  Pbase=100e6  Vbase=500e3  OutputType=Complex  PhasorSimulation=off  PSBequivalent=0
  BUS-89 : spsThreePhaseVIMeasurementLib/Three-Phase V-I Measurement  VoltageMeasurement=phase-to-phase  SetLabelV=on  LabelV=V_ll_89  Vpu=off  VpuLL=off  CurrentMeasurement=yes  SetLabelI=on  LabelI=I_89  Ipu=off  Pbase=100e6  Vbase=500e3  OutputType=Complex  PhasorSimulation=off  PSBequivalent=0
  BUS-90 : spsThreePhaseVIMeasurementLib/Three-Phase V-I Measurement  VoltageMeasurement=phase-to-phase  SetLabelV=on  LabelV=V_ll_90  Vpu=off  VpuLL=off  CurrentMeasurement=yes  SetLabelI=on  LabelI=I_90  Ipu=off  Pbase=100e6  Vbase=500e3  OutputType=Complex  PhasorSimulation=off  PSBequivalent=0
  BUS-91 : spsThreePhaseVIMeasurementLib/Three-Phase V-I Measurement  VoltageMeasurement=phase-to-phase  SetLabelV=on  LabelV=V_ll_91  Vpu=off  VpuLL=off  CurrentMeasurement=yes  SetLabelI=on  LabelI=I_91  Ipu=off  Pbase=100e6  Vbase=500e3  OutputType=Complex  PhasorSimulation=off  PSBequivalent=0
  BUS-92 : spsThreePhaseVIMeasurementLib/Three-Phase V-I Measurement  VoltageMeasurement=phase-to-phase  SetLabelV=on  LabelV=V_ll_92  Vpu=off  VpuLL=off  CurrentMeasurement=yes  SetLabelI=on  LabelI=I_92  Ipu=off  Pbase=100e6  Vbase=500e3  OutputType=Complex  PhasorSimulation=off  PSBequivalent=0
  BUS-93 : spsThreePhaseVIMeasurementLib/Three-Phase V-I Measurement  VoltageMeasurement=phase-to-phase  SetLabelV=on  LabelV=V_ll_93  Vpu=off  VpuLL=off  CurrentMeasurement=yes  SetLabelI=on  LabelI=I_93  Ipu=off  Pbase=100e6  Vbase=500e3  OutputType=Complex  PhasorSimulation=off  PSBequivalent=0
  BUS-94 : spsThreePhaseVIMeasurementLib/Three-Phase V-I Measurement  VoltageMeasurement=phase-to-phase  SetLabelV=on  LabelV=V_ll_94  Vpu=off  VpuLL=off  CurrentMeasurement=yes  SetLabelI=on  LabelI=I_94  Ipu=off  Pbase=100e6  Vbase=500e3  OutputType=Complex  PhasorSimulation=off  PSBequivalent=0
  BUS-95 : spsThreePhaseVIMeasurementLib/Three-Phase V-I Measurement  VoltageMeasurement=phase-to-phase  SetLabelV=on  LabelV=V_ll_95  Vpu=off  VpuLL=off  CurrentMeasurement=yes  SetLabelI=on  LabelI=I_95  Ipu=off  Pbase=100e6  Vbase=500e3  OutputType=Complex  PhasorSimulation=off  PSBequivalent=0
  BUS-96 : spsThreePhaseVIMeasurementLib/Three-Phase V-I Measurement  VoltageMeasurement=phase-to-phase  SetLabelV=on  LabelV=V_ll_96  Vpu=off  VpuLL=off  CurrentMeasurement=yes  SetLabelI=on  LabelI=I_96  Ipu=off  Pbase=100e6  Vbase=500e3  OutputType=Complex  PhasorSimulation=off  PSBequivalent=0
  BUS-97 : spsThreePhaseVIMeasurementLib/Three-Phase V-I Measurement  VoltageMeasurement=phase-to-phase  SetLabelV=on  LabelV=V_ll_97  Vpu=off  VpuLL=off  CurrentMeasurement=yes  SetLabelI=on  LabelI=I_97  Ipu=off  Pbase=100e6  Vbase=500e3  OutputType=Complex  PhasorSimulation=off  PSBequivalent=0
  BUS-98 : spsThreePhaseVIMeasurementLib/Three-Phase V-I Measurement  VoltageMeasurement=phase-to-phase  SetLabelV=on  LabelV=V_ll_98  Vpu=off  VpuLL=off  CurrentMeasurement=yes  SetLabelI=on  LabelI=I_98  Ipu=off  Pbase=100e6  Vbase=500e3  OutputType=Complex  PhasorSimulation=off  PSBequivalent=0
  BUS-99 : spsThreePhaseVIMeasurementLib/Three-Phase V-I Measurement  VoltageMeasurement=phase-to-phase  SetLabelV=on  LabelV=V_ll_99  Vpu=off  VpuLL=off  CurrentMeasurement=yes  SetLabelI=on  LabelI=I_99  Ipu=off  Pbase=100e6  Vbase=500e3  OutputType=Complex  PhasorSimulation=off  PSBequivalent=0
  BUS-Load-1 : spsThreePhaseVIMeasurementLib/Three-Phase V-I Measurement  VoltageMeasurement=phase-to-phase  SetLabelV=on  LabelV=V_Load_1  Vpu=off  VpuLL=off  CurrentMeasurement=yes  SetLabelI=on  LabelI=I_Load1  Ipu=off  Pbase=100e6  Vbase=500e3  OutputType=Complex  PhasorSimulation=off  PSBequivalent=0
  BUS-Load-10 : spsThreePhaseVIMeasurementLib/Three-Phase V-I Measurement  VoltageMeasurement=phase-to-phase  SetLabelV=on  LabelV=V_Load_10  Vpu=off  VpuLL=off  CurrentMeasurement=yes  SetLabelI=on  LabelI=I_Load10  Ipu=off  Pbase=100e6  Vbase=500e3  OutputType=Complex  PhasorSimulation=off  PSBequivalent=0
  BUS-Load-11 : spsThreePhaseVIMeasurementLib/Three-Phase V-I Measurement  VoltageMeasurement=phase-to-phase  SetLabelV=on  LabelV=V_Load_11  Vpu=off  VpuLL=off  CurrentMeasurement=yes  SetLabelI=on  LabelI=I_Load11  Ipu=off  Pbase=100e6  Vbase=500e3  OutputType=Complex  PhasorSimulation=off  PSBequivalent=0
  BUS-Load-12 : spsThreePhaseVIMeasurementLib/Three-Phase V-I Measurement  VoltageMeasurement=phase-to-phase  SetLabelV=on  LabelV=V_Load_12  Vpu=off  VpuLL=off  CurrentMeasurement=yes  SetLabelI=on  LabelI=I_Load12  Ipu=off  Pbase=100e6  Vbase=500e3  OutputType=Complex  PhasorSimulation=off  PSBequivalent=0
  BUS-Load-13 : spsThreePhaseVIMeasurementLib/Three-Phase V-I Measurement  VoltageMeasurement=phase-to-phase  SetLabelV=on  LabelV=V_Load_13  Vpu=off  VpuLL=off  CurrentMeasurement=yes  SetLabelI=on  LabelI=I_Load13  Ipu=off  Pbase=100e6  Vbase=500e3  OutputType=Complex  PhasorSimulation=off  PSBequivalent=0
  BUS-Load-14 : spsThreePhaseVIMeasurementLib/Three-Phase V-I Measurement  VoltageMeasurement=phase-to-phase  SetLabelV=on  LabelV=V_Load_14  Vpu=off  VpuLL=off  CurrentMeasurement=yes  SetLabelI=on  LabelI=I_Load14  Ipu=off  Pbase=100e6  Vbase=500e3  OutputType=Complex  PhasorSimulation=off  PSBequivalent=0
  BUS-Load-15 : spsThreePhaseVIMeasurementLib/Three-Phase V-I Measurement  VoltageMeasurement=phase-to-phase  SetLabelV=on  LabelV=V_Load_15  Vpu=off  VpuLL=off  CurrentMeasurement=yes  SetLabelI=on  LabelI=I_Load15  Ipu=off  Pbase=100e6  Vbase=500e3  OutputType=Complex  PhasorSimulation=off  PSBequivalent=0
  BUS-Load-16 : spsThreePhaseVIMeasurementLib/Three-Phase V-I Measurement  VoltageMeasurement=phase-to-phase  SetLabelV=on  LabelV=V_Load_16  Vpu=off  VpuLL=off  CurrentMeasurement=yes  SetLabelI=on  LabelI=I_Load16  Ipu=off  Pbase=100e6  Vbase=500e3  OutputType=Complex  PhasorSimulation=off  PSBequivalent=0
  BUS-Load-17 : spsThreePhaseVIMeasurementLib/Three-Phase V-I Measurement  VoltageMeasurement=phase-to-phase  SetLabelV=on  LabelV=V_Load_17  Vpu=off  VpuLL=off  CurrentMeasurement=yes  SetLabelI=on  LabelI=I_Load17  Ipu=off  Pbase=100e6  Vbase=500e3  OutputType=Complex  PhasorSimulation=off  PSBequivalent=0
  BUS-Load-18 : spsThreePhaseVIMeasurementLib/Three-Phase V-I Measurement  VoltageMeasurement=phase-to-phase  SetLabelV=on  LabelV=V_Load_18  Vpu=off  VpuLL=off  CurrentMeasurement=yes  SetLabelI=on  LabelI=I_Load18  Ipu=off  Pbase=100e6  Vbase=500e3  OutputType=Complex  PhasorSimulation=off  PSBequivalent=0
  BUS-Load-19 : spsThreePhaseVIMeasurementLib/Three-Phase V-I Measurement  VoltageMeasurement=phase-to-phase  SetLabelV=on  LabelV=V_Load_19  Vpu=off  VpuLL=off  CurrentMeasurement=yes  SetLabelI=on  LabelI=I_Load19  Ipu=off  Pbase=100e6  Vbase=500e3  OutputType=Complex  PhasorSimulation=off  PSBequivalent=0
  BUS-Load-2 : spsThreePhaseVIMeasurementLib/Three-Phase V-I Measurement  VoltageMeasurement=phase-to-phase  SetLabelV=on  LabelV=V_Load_2  Vpu=off  VpuLL=off  CurrentMeasurement=yes  SetLabelI=on  LabelI=I_Load2  Ipu=off  Pbase=100e6  Vbase=500e3  OutputType=Complex  PhasorSimulation=off  PSBequivalent=0
  BUS-Load-20 : spsThreePhaseVIMeasurementLib/Three-Phase V-I Measurement  VoltageMeasurement=phase-to-phase  SetLabelV=on  LabelV=V_Load_20  Vpu=off  VpuLL=off  CurrentMeasurement=yes  SetLabelI=on  LabelI=I_Load20  Ipu=off  Pbase=100e6  Vbase=500e3  OutputType=Complex  PhasorSimulation=off  PSBequivalent=0
  BUS-Load-21 : spsThreePhaseVIMeasurementLib/Three-Phase V-I Measurement  VoltageMeasurement=phase-to-phase  SetLabelV=on  LabelV=V_Load_21  Vpu=off  VpuLL=off  CurrentMeasurement=yes  SetLabelI=on  LabelI=I_Load21  Ipu=off  Pbase=100e6  Vbase=500e3  OutputType=Complex  PhasorSimulation=off  PSBequivalent=0
  BUS-Load-22 : spsThreePhaseVIMeasurementLib/Three-Phase V-I Measurement  VoltageMeasurement=phase-to-phase  SetLabelV=on  LabelV=V_Load_22  Vpu=off  VpuLL=off  CurrentMeasurement=yes  SetLabelI=on  LabelI=I_Load22  Ipu=off  Pbase=100e6  Vbase=500e3  OutputType=Complex  PhasorSimulation=off  PSBequivalent=0
  BUS-Load-23 : spsThreePhaseVIMeasurementLib/Three-Phase V-I Measurement  VoltageMeasurement=phase-to-phase  SetLabelV=on  LabelV=V_Load_23  Vpu=off  VpuLL=off  CurrentMeasurement=yes  SetLabelI=on  LabelI=I_Load23  Ipu=off  Pbase=100e6  Vbase=500e3  OutputType=Complex  PhasorSimulation=off  PSBequivalent=0
  BUS-Load-24 : spsThreePhaseVIMeasurementLib/Three-Phase V-I Measurement  VoltageMeasurement=phase-to-phase  SetLabelV=on  LabelV=V_Load_24  Vpu=off  VpuLL=off  CurrentMeasurement=yes  SetLabelI=on  LabelI=I_Load24  Ipu=off  Pbase=100e6  Vbase=500e3  OutputType=Complex  PhasorSimulation=off  PSBequivalent=0
  BUS-Load-25 : spsThreePhaseVIMeasurementLib/Three-Phase V-I Measurement  VoltageMeasurement=phase-to-phase  SetLabelV=on  LabelV=V_Load_25  Vpu=off  VpuLL=off  CurrentMeasurement=yes  SetLabelI=on  LabelI=I_Load25  Ipu=off  Pbase=100e6  Vbase=500e3  OutputType=Complex  PhasorSimulation=off  PSBequivalent=0
  BUS-Load-26 : spsThreePhaseVIMeasurementLib/Three-Phase V-I Measurement  VoltageMeasurement=phase-to-phase  SetLabelV=on  LabelV=V_Load_26  Vpu=off  VpuLL=off  CurrentMeasurement=yes  SetLabelI=on  LabelI=I_Load26  Ipu=off  Pbase=100e6  Vbase=500e3  OutputType=Complex  PhasorSimulation=off  PSBequivalent=0
  BUS-Load-27 : spsThreePhaseVIMeasurementLib/Three-Phase V-I Measurement  VoltageMeasurement=phase-to-phase  SetLabelV=on  LabelV=V_Load_27  Vpu=off  VpuLL=off  CurrentMeasurement=yes  SetLabelI=on  LabelI=I_Load27  Ipu=off  Pbase=100e6  Vbase=500e3  OutputType=Complex  PhasorSimulation=off  PSBequivalent=0
  BUS-Load-28 : spsThreePhaseVIMeasurementLib/Three-Phase V-I Measurement  VoltageMeasurement=phase-to-phase  SetLabelV=on  LabelV=V_Load_28  Vpu=off  VpuLL=off  CurrentMeasurement=yes  SetLabelI=on  LabelI=I_Load28  Ipu=off  Pbase=100e6  Vbase=500e3  OutputType=Complex  PhasorSimulation=off  PSBequivalent=0
  BUS-Load-29 : spsThreePhaseVIMeasurementLib/Three-Phase V-I Measurement  VoltageMeasurement=phase-to-phase  SetLabelV=on  LabelV=V_Load_29  Vpu=off  VpuLL=off  CurrentMeasurement=yes  SetLabelI=on  LabelI=I_Load29  Ipu=off  Pbase=100e6  Vbase=500e3  OutputType=Complex  PhasorSimulation=off  PSBequivalent=0
  BUS-Load-3 : spsThreePhaseVIMeasurementLib/Three-Phase V-I Measurement  VoltageMeasurement=phase-to-phase  SetLabelV=on  LabelV=V_Load_3  Vpu=off  VpuLL=off  CurrentMeasurement=yes  SetLabelI=on  LabelI=I_Load3  Ipu=off  Pbase=100e6  Vbase=500e3  OutputType=Complex  PhasorSimulation=off  PSBequivalent=0
  BUS-Load-30 : spsThreePhaseVIMeasurementLib/Three-Phase V-I Measurement  VoltageMeasurement=phase-to-phase  SetLabelV=on  LabelV=V_Load_30  Vpu=off  VpuLL=off  CurrentMeasurement=yes  SetLabelI=on  LabelI=I_Load30  Ipu=off  Pbase=100e6  Vbase=500e3  OutputType=Complex  PhasorSimulation=off  PSBequivalent=0
  BUS-Load-31 : spsThreePhaseVIMeasurementLib/Three-Phase V-I Measurement  VoltageMeasurement=phase-to-phase  SetLabelV=on  LabelV=V_Load_31  Vpu=off  VpuLL=off  CurrentMeasurement=yes  SetLabelI=on  LabelI=I_Load31  Ipu=off  Pbase=100e6  Vbase=500e3  OutputType=Complex  PhasorSimulation=off  PSBequivalent=0
  BUS-Load-32 : spsThreePhaseVIMeasurementLib/Three-Phase V-I Measurement  VoltageMeasurement=phase-to-phase  SetLabelV=on  LabelV=V_Load_32  Vpu=off  VpuLL=off  CurrentMeasurement=yes  SetLabelI=on  LabelI=I_Load32  Ipu=off  Pbase=100e6  Vbase=500e3  OutputType=Complex  PhasorSimulation=off  PSBequivalent=0
  BUS-Load-33 : spsThreePhaseVIMeasurementLib/Three-Phase V-I Measurement  VoltageMeasurement=phase-to-phase  SetLabelV=on  LabelV=V_Load_33  Vpu=off  VpuLL=off  CurrentMeasurement=yes  SetLabelI=on  LabelI=I_Load33  Ipu=off  Pbase=100e6  Vbase=500e3  OutputType=Complex  PhasorSimulation=off  PSBequivalent=0
  BUS-Load-34 : spsThreePhaseVIMeasurementLib/Three-Phase V-I Measurement  VoltageMeasurement=phase-to-phase  SetLabelV=on  LabelV=V_Load_34  Vpu=off  VpuLL=off  CurrentMeasurement=yes  SetLabelI=on  LabelI=I_Load34  Ipu=off  Pbase=100e6  Vbase=500e3  OutputType=Complex  PhasorSimulation=off  PSBequivalent=0
  BUS-Load-35 : spsThreePhaseVIMeasurementLib/Three-Phase V-I Measurement  VoltageMeasurement=phase-to-phase  SetLabelV=on  LabelV=V_Load_35  Vpu=off  VpuLL=off  CurrentMeasurement=yes  SetLabelI=on  LabelI=I_Load35  Ipu=off  Pbase=100e6  Vbase=500e3  OutputType=Complex  PhasorSimulation=off  PSBequivalent=0
  BUS-Load-36 : spsThreePhaseVIMeasurementLib/Three-Phase V-I Measurement  VoltageMeasurement=phase-to-phase  SetLabelV=on  LabelV=V_Load_36  Vpu=off  VpuLL=off  CurrentMeasurement=yes  SetLabelI=on  LabelI=I_Load36  Ipu=off  Pbase=100e6  Vbase=500e3  OutputType=Complex  PhasorSimulation=off  PSBequivalent=0
  BUS-Load-37 : spsThreePhaseVIMeasurementLib/Three-Phase V-I Measurement  VoltageMeasurement=phase-to-phase  SetLabelV=on  LabelV=V_Load_37  Vpu=off  VpuLL=off  CurrentMeasurement=yes  SetLabelI=on  LabelI=I_Load37  Ipu=off  Pbase=100e6  Vbase=500e3  OutputType=Complex  PhasorSimulation=off  PSBequivalent=0
  BUS-Load-38 : spsThreePhaseVIMeasurementLib/Three-Phase V-I Measurement  VoltageMeasurement=phase-to-phase  SetLabelV=on  LabelV=V_Load_38  Vpu=off  VpuLL=off  CurrentMeasurement=yes  SetLabelI=on  LabelI=I_Load38  Ipu=off  Pbase=100e6  Vbase=500e3  OutputType=Complex  PhasorSimulation=off  PSBequivalent=0
  BUS-Load-39 : spsThreePhaseVIMeasurementLib/Three-Phase V-I Measurement  VoltageMeasurement=phase-to-phase  SetLabelV=on  LabelV=V_Load_39  Vpu=off  VpuLL=off  CurrentMeasurement=yes  SetLabelI=on  LabelI=I_Load39  Ipu=off  Pbase=100e6  Vbase=500e3  OutputType=Complex  PhasorSimulation=off  PSBequivalent=0
  BUS-Load-4 : spsThreePhaseVIMeasurementLib/Three-Phase V-I Measurement  VoltageMeasurement=phase-to-phase  SetLabelV=on  LabelV=V_Load_4  Vpu=off  VpuLL=off  CurrentMeasurement=yes  SetLabelI=on  LabelI=I_Load4  Ipu=off  Pbase=100e6  Vbase=500e3  OutputType=Complex  PhasorSimulation=off  PSBequivalent=0
  BUS-Load-40 : spsThreePhaseVIMeasurementLib/Three-Phase V-I Measurement  VoltageMeasurement=phase-to-phase  SetLabelV=on  LabelV=V_Load_40  Vpu=off  VpuLL=off  CurrentMeasurement=yes  SetLabelI=on  LabelI=I_Load40  Ipu=off  Pbase=100e6  Vbase=500e3  OutputType=Complex  PhasorSimulation=off  PSBequivalent=0
  BUS-Load-41 : spsThreePhaseVIMeasurementLib/Three-Phase V-I Measurement  VoltageMeasurement=phase-to-phase  SetLabelV=on  LabelV=V_Load_41  Vpu=off  VpuLL=off  CurrentMeasurement=yes  SetLabelI=on  LabelI=I_Load41  Ipu=off  Pbase=100e6  Vbase=500e3  OutputType=Complex  PhasorSimulation=off  PSBequivalent=0
  BUS-Load-42 : spsThreePhaseVIMeasurementLib/Three-Phase V-I Measurement  VoltageMeasurement=phase-to-phase  SetLabelV=on  LabelV=V_Load_42  Vpu=off  VpuLL=off  CurrentMeasurement=yes  SetLabelI=on  LabelI=I_Load42  Ipu=off  Pbase=100e6  Vbase=500e3  OutputType=Complex  PhasorSimulation=off  PSBequivalent=0
  BUS-Load-43 : spsThreePhaseVIMeasurementLib/Three-Phase V-I Measurement  VoltageMeasurement=phase-to-phase  SetLabelV=on  LabelV=V_Load_43  Vpu=off  VpuLL=off  CurrentMeasurement=yes  SetLabelI=on  LabelI=I_Load43  Ipu=off  Pbase=100e6  Vbase=500e3  OutputType=Complex  PhasorSimulation=off  PSBequivalent=0
  BUS-Load-44 : spsThreePhaseVIMeasurementLib/Three-Phase V-I Measurement  VoltageMeasurement=phase-to-phase  SetLabelV=on  LabelV=V_Load_44  Vpu=off  VpuLL=off  CurrentMeasurement=yes  SetLabelI=on  LabelI=I_Load44  Ipu=off  Pbase=100e6  Vbase=500e3  OutputType=Complex  PhasorSimulation=off  PSBequivalent=0
  BUS-Load-45 : spsThreePhaseVIMeasurementLib/Three-Phase V-I Measurement  VoltageMeasurement=phase-to-phase  SetLabelV=on  LabelV=V_Load_45  Vpu=off  VpuLL=off  CurrentMeasurement=yes  SetLabelI=on  LabelI=I_Load45  Ipu=off  Pbase=100e6  Vbase=500e3  OutputType=Complex  PhasorSimulation=off  PSBequivalent=0
  BUS-Load-46 : spsThreePhaseVIMeasurementLib/Three-Phase V-I Measurement  VoltageMeasurement=phase-to-phase  SetLabelV=on  LabelV=V_Load_46  Vpu=off  VpuLL=off  CurrentMeasurement=yes  SetLabelI=on  LabelI=I_Load46  Ipu=off  Pbase=100e6  Vbase=500e3  OutputType=Complex  PhasorSimulation=off  PSBequivalent=0
  BUS-Load-47 : spsThreePhaseVIMeasurementLib/Three-Phase V-I Measurement  VoltageMeasurement=phase-to-phase  SetLabelV=on  LabelV=V_Load_47  Vpu=off  VpuLL=off  CurrentMeasurement=yes  SetLabelI=on  LabelI=I_Load47  Ipu=off  Pbase=100e6  Vbase=500e3  OutputType=Complex  PhasorSimulation=off  PSBequivalent=0
  BUS-Load-48 : spsThreePhaseVIMeasurementLib/Three-Phase V-I Measurement  VoltageMeasurement=phase-to-phase  SetLabelV=on  LabelV=V_Load_48  Vpu=off  VpuLL=off  CurrentMeasurement=yes  SetLabelI=on  LabelI=I_Load48  Ipu=off  Pbase=100e6  Vbase=500e3  OutputType=Complex  PhasorSimulation=off  PSBequivalent=0
  BUS-Load-49 : spsThreePhaseVIMeasurementLib/Three-Phase V-I Measurement  VoltageMeasurement=phase-to-phase  SetLabelV=on  LabelV=V_Load_49  Vpu=off  VpuLL=off  CurrentMeasurement=yes  SetLabelI=on  LabelI=I_Load49  Ipu=off  Pbase=100e6  Vbase=500e3  OutputType=Complex  PhasorSimulation=off  PSBequivalent=0
  BUS-Load-5 : spsThreePhaseVIMeasurementLib/Three-Phase V-I Measurement  VoltageMeasurement=phase-to-phase  SetLabelV=on  LabelV=V_Load_5  Vpu=off  VpuLL=off  CurrentMeasurement=yes  SetLabelI=on  LabelI=I_Load5  Ipu=off  Pbase=100e6  Vbase=500e3  OutputType=Complex  PhasorSimulation=off  PSBequivalent=0
  BUS-Load-50 : spsThreePhaseVIMeasurementLib/Three-Phase V-I Measurement  VoltageMeasurement=phase-to-phase  SetLabelV=on  LabelV=V_Load_50  Vpu=off  VpuLL=off  CurrentMeasurement=yes  SetLabelI=on  LabelI=I_Load50  Ipu=off  Pbase=100e6  Vbase=500e3  OutputType=Complex  PhasorSimulation=off  PSBequivalent=0
  BUS-Load-51 : spsThreePhaseVIMeasurementLib/Three-Phase V-I Measurement  VoltageMeasurement=phase-to-phase  SetLabelV=on  LabelV=V_Load_51  Vpu=off  VpuLL=off  CurrentMeasurement=yes  SetLabelI=on  LabelI=I_Load51  Ipu=off  Pbase=100e6  Vbase=500e3  OutputType=Complex  PhasorSimulation=off  PSBequivalent=0
  BUS-Load-52 : spsThreePhaseVIMeasurementLib/Three-Phase V-I Measurement  VoltageMeasurement=phase-to-phase  SetLabelV=on  LabelV=V_Load_52  Vpu=off  VpuLL=off  CurrentMeasurement=yes  SetLabelI=on  LabelI=I_Load52  Ipu=off  Pbase=100e6  Vbase=500e3  OutputType=Complex  PhasorSimulation=off  PSBequivalent=0
  BUS-Load-53 : spsThreePhaseVIMeasurementLib/Three-Phase V-I Measurement  VoltageMeasurement=phase-to-phase  SetLabelV=on  LabelV=V_Load_53  Vpu=off  VpuLL=off  CurrentMeasurement=yes  SetLabelI=on  LabelI=I_Load53  Ipu=off  Pbase=100e6  Vbase=500e3  OutputType=Complex  PhasorSimulation=off  PSBequivalent=0
  BUS-Load-54 : spsThreePhaseVIMeasurementLib/Three-Phase V-I Measurement  VoltageMeasurement=phase-to-phase  SetLabelV=on  LabelV=V_Load_54  Vpu=off  VpuLL=off  CurrentMeasurement=yes  SetLabelI=on  LabelI=I_Load54  Ipu=off  Pbase=100e6  Vbase=500e3  OutputType=Complex  PhasorSimulation=off  PSBequivalent=0
  BUS-Load-55 : spsThreePhaseVIMeasurementLib/Three-Phase V-I Measurement  VoltageMeasurement=phase-to-phase  SetLabelV=on  LabelV=V_Load_55  Vpu=off  VpuLL=off  CurrentMeasurement=yes  SetLabelI=on  LabelI=I_Load55  Ipu=off  Pbase=100e6  Vbase=500e3  OutputType=Complex  PhasorSimulation=off  PSBequivalent=0
  BUS-Load-56 : spsThreePhaseVIMeasurementLib/Three-Phase V-I Measurement  VoltageMeasurement=phase-to-phase  SetLabelV=on  LabelV=V_Load_56  Vpu=off  VpuLL=off  CurrentMeasurement=yes  SetLabelI=on  LabelI=I_Load56  Ipu=off  Pbase=100e6  Vbase=500e3  OutputType=Complex  PhasorSimulation=off  PSBequivalent=0
  BUS-Load-57 : spsThreePhaseVIMeasurementLib/Three-Phase V-I Measurement  VoltageMeasurement=phase-to-phase  SetLabelV=on  LabelV=V_Load_57  Vpu=off  VpuLL=off  CurrentMeasurement=yes  SetLabelI=on  LabelI=I_Load57  Ipu=off  Pbase=100e6  Vbase=500e3  OutputType=Complex  PhasorSimulation=off  PSBequivalent=0
  BUS-Load-58 : spsThreePhaseVIMeasurementLib/Three-Phase V-I Measurement  VoltageMeasurement=phase-to-phase  SetLabelV=on  LabelV=V_Load_58  Vpu=off  VpuLL=off  CurrentMeasurement=yes  SetLabelI=on  LabelI=I_Load58  Ipu=off  Pbase=100e6  Vbase=500e3  OutputType=Complex  PhasorSimulation=off  PSBequivalent=0
  BUS-Load-59 : spsThreePhaseVIMeasurementLib/Three-Phase V-I Measurement  VoltageMeasurement=phase-to-phase  SetLabelV=on  LabelV=V_Load_59  Vpu=off  VpuLL=off  CurrentMeasurement=yes  SetLabelI=on  LabelI=I_Load59  Ipu=off  Pbase=100e6  Vbase=500e3  OutputType=Complex  PhasorSimulation=off  PSBequivalent=0
  BUS-Load-6 : spsThreePhaseVIMeasurementLib/Three-Phase V-I Measurement  VoltageMeasurement=phase-to-phase  SetLabelV=on  LabelV=V_Load_6  Vpu=off  VpuLL=off  CurrentMeasurement=yes  SetLabelI=on  LabelI=I_Load6  Ipu=off  Pbase=100e6  Vbase=500e3  OutputType=Complex  PhasorSimulation=off  PSBequivalent=0
  BUS-Load-60 : spsThreePhaseVIMeasurementLib/Three-Phase V-I Measurement  VoltageMeasurement=phase-to-phase  SetLabelV=on  LabelV=V_Load_60  Vpu=off  VpuLL=off  CurrentMeasurement=yes  SetLabelI=on  LabelI=I_Load60  Ipu=off  Pbase=100e6  Vbase=500e3  OutputType=Complex  PhasorSimulation=off  PSBequivalent=0
  BUS-Load-61 : spsThreePhaseVIMeasurementLib/Three-Phase V-I Measurement  VoltageMeasurement=phase-to-phase  SetLabelV=on  LabelV=V_Load_61  Vpu=off  VpuLL=off  CurrentMeasurement=yes  SetLabelI=on  LabelI=I_Load61  Ipu=off  Pbase=100e6  Vbase=500e3  OutputType=Complex  PhasorSimulation=off  PSBequivalent=0
  BUS-Load-62 : spsThreePhaseVIMeasurementLib/Three-Phase V-I Measurement  VoltageMeasurement=phase-to-phase  SetLabelV=on  LabelV=V_Load_62  Vpu=off  VpuLL=off  CurrentMeasurement=yes  SetLabelI=on  LabelI=I_Load62  Ipu=off  Pbase=100e6  Vbase=500e3  OutputType=Complex  PhasorSimulation=off  PSBequivalent=0
  BUS-Load-63 : spsThreePhaseVIMeasurementLib/Three-Phase V-I Measurement  VoltageMeasurement=phase-to-phase  SetLabelV=on  LabelV=V_Load_63  Vpu=off  VpuLL=off  CurrentMeasurement=yes  SetLabelI=on  LabelI=I_Load63  Ipu=off  Pbase=100e6  Vbase=500e3  OutputType=Complex  PhasorSimulation=off  PSBequivalent=0
  BUS-Load-64 : spsThreePhaseVIMeasurementLib/Three-Phase V-I Measurement  VoltageMeasurement=phase-to-phase  SetLabelV=on  LabelV=V_Load_64  Vpu=off  VpuLL=off  CurrentMeasurement=yes  SetLabelI=on  LabelI=I_Load64  Ipu=off  Pbase=100e6  Vbase=500e3  OutputType=Complex  PhasorSimulation=off  PSBequivalent=0
  BUS-Load-65 : spsThreePhaseVIMeasurementLib/Three-Phase V-I Measurement  VoltageMeasurement=phase-to-phase  SetLabelV=on  LabelV=V_Load_65  Vpu=off  VpuLL=off  CurrentMeasurement=yes  SetLabelI=on  LabelI=I_Load65  Ipu=off  Pbase=100e6  Vbase=500e3  OutputType=Complex  PhasorSimulation=off  PSBequivalent=0
  BUS-Load-66 : spsThreePhaseVIMeasurementLib/Three-Phase V-I Measurement  VoltageMeasurement=phase-to-phase  SetLabelV=on  LabelV=V_Load_66  Vpu=off  VpuLL=off  CurrentMeasurement=yes  SetLabelI=on  LabelI=I_Load66  Ipu=off  Pbase=100e6  Vbase=500e3  OutputType=Complex  PhasorSimulation=off  PSBequivalent=0
  BUS-Load-67 : spsThreePhaseVIMeasurementLib/Three-Phase V-I Measurement  VoltageMeasurement=phase-to-phase  SetLabelV=on  LabelV=V_Load_67  Vpu=off  VpuLL=off  CurrentMeasurement=yes  SetLabelI=on  LabelI=I_Load67  Ipu=off  Pbase=100e6  Vbase=500e3  OutputType=Complex  PhasorSimulation=off  PSBequivalent=0
  BUS-Load-68 : spsThreePhaseVIMeasurementLib/Three-Phase V-I Measurement  VoltageMeasurement=phase-to-phase  SetLabelV=on  LabelV=V_Load_68  Vpu=off  VpuLL=off  CurrentMeasurement=yes  SetLabelI=on  LabelI=I_Load68  Ipu=off  Pbase=100e6  Vbase=500e3  OutputType=Complex  PhasorSimulation=off  PSBequivalent=0
  BUS-Load-69 : spsThreePhaseVIMeasurementLib/Three-Phase V-I Measurement  VoltageMeasurement=phase-to-phase  SetLabelV=on  LabelV=V_Load_69  Vpu=off  VpuLL=off  CurrentMeasurement=yes  SetLabelI=on  LabelI=I_Load69  Ipu=off  Pbase=100e6  Vbase=500e3  OutputType=Complex  PhasorSimulation=off  PSBequivalent=0
  BUS-Load-7 : spsThreePhaseVIMeasurementLib/Three-Phase V-I Measurement  VoltageMeasurement=phase-to-phase  SetLabelV=on  LabelV=V_Load_7  Vpu=off  VpuLL=off  CurrentMeasurement=yes  SetLabelI=on  LabelI=I_Load7  Ipu=off  Pbase=100e6  Vbase=500e3  OutputType=Complex  PhasorSimulation=off  PSBequivalent=0
  BUS-Load-70 : spsThreePhaseVIMeasurementLib/Three-Phase V-I Measurement  VoltageMeasurement=phase-to-phase  SetLabelV=on  LabelV=V_Load_70  Vpu=off  VpuLL=off  CurrentMeasurement=yes  SetLabelI=on  LabelI=I_Load70  Ipu=off  Pbase=100e6  Vbase=500e3  OutputType=Complex  PhasorSimulation=off  PSBequivalent=0
  BUS-Load-71 : spsThreePhaseVIMeasurementLib/Three-Phase V-I Measurement  VoltageMeasurement=phase-to-phase  SetLabelV=on  LabelV=V_Load_71  Vpu=off  VpuLL=off  CurrentMeasurement=yes  SetLabelI=on  LabelI=I_Load71  Ipu=off  Pbase=100e6  Vbase=500e3  OutputType=Complex  PhasorSimulation=off  PSBequivalent=0
  BUS-Load-72 : spsThreePhaseVIMeasurementLib/Three-Phase V-I Measurement  VoltageMeasurement=phase-to-phase  SetLabelV=on  LabelV=V_Load_72  Vpu=off  VpuLL=off  CurrentMeasurement=yes  SetLabelI=on  LabelI=I_Load72  Ipu=off  Pbase=100e6  Vbase=500e3  OutputType=Complex  PhasorSimulation=off  PSBequivalent=0
  BUS-Load-73 : spsThreePhaseVIMeasurementLib/Three-Phase V-I Measurement  VoltageMeasurement=phase-to-phase  SetLabelV=on  LabelV=V_Load_73  Vpu=off  VpuLL=off  CurrentMeasurement=yes  SetLabelI=on  LabelI=I_Load73  Ipu=off  Pbase=100e6  Vbase=500e3  OutputType=Complex  PhasorSimulation=off  PSBequivalent=0
  BUS-Load-74 : spsThreePhaseVIMeasurementLib/Three-Phase V-I Measurement  VoltageMeasurement=phase-to-phase  SetLabelV=on  LabelV=V_Load_74  Vpu=off  VpuLL=off  CurrentMeasurement=yes  SetLabelI=on  LabelI=I_Load74  Ipu=off  Pbase=100e6  Vbase=500e3  OutputType=Complex  PhasorSimulation=off  PSBequivalent=0
  BUS-Load-75 : spsThreePhaseVIMeasurementLib/Three-Phase V-I Measurement  VoltageMeasurement=phase-to-phase  SetLabelV=on  LabelV=V_Load_75  Vpu=off  VpuLL=off  CurrentMeasurement=yes  SetLabelI=on  LabelI=I_Load75  Ipu=off  Pbase=100e6  Vbase=500e3  OutputType=Complex  PhasorSimulation=off  PSBequivalent=0
  BUS-Load-76 : spsThreePhaseVIMeasurementLib/Three-Phase V-I Measurement  VoltageMeasurement=phase-to-phase  SetLabelV=on  LabelV=V_Load_76  Vpu=off  VpuLL=off  CurrentMeasurement=yes  SetLabelI=on  LabelI=I_Load76  Ipu=off  Pbase=100e6  Vbase=500e3  OutputType=Complex  PhasorSimulation=off  PSBequivalent=0
  BUS-Load-77 : spsThreePhaseVIMeasurementLib/Three-Phase V-I Measurement  VoltageMeasurement=phase-to-phase  SetLabelV=on  LabelV=V_Load_77  Vpu=off  VpuLL=off  CurrentMeasurement=yes  SetLabelI=on  LabelI=I_Load77  Ipu=off  Pbase=100e6  Vbase=500e3  OutputType=Complex  PhasorSimulation=off  PSBequivalent=0
  BUS-Load-78 : spsThreePhaseVIMeasurementLib/Three-Phase V-I Measurement  VoltageMeasurement=phase-to-phase  SetLabelV=on  LabelV=V_Load_78  Vpu=off  VpuLL=off  CurrentMeasurement=yes  SetLabelI=on  LabelI=I_Load78  Ipu=off  Pbase=100e6  Vbase=500e3  OutputType=Complex  PhasorSimulation=off  PSBequivalent=0
  BUS-Load-79 : spsThreePhaseVIMeasurementLib/Three-Phase V-I Measurement  VoltageMeasurement=phase-to-phase  SetLabelV=on  LabelV=V_Load_79  Vpu=off  VpuLL=off  CurrentMeasurement=yes  SetLabelI=on  LabelI=I_Load79  Ipu=off  Pbase=100e6  Vbase=500e3  OutputType=Complex  PhasorSimulation=off  PSBequivalent=0
  BUS-Load-8 : spsThreePhaseVIMeasurementLib/Three-Phase V-I Measurement  VoltageMeasurement=phase-to-phase  SetLabelV=on  LabelV=V_Load_8  Vpu=off  VpuLL=off  CurrentMeasurement=yes  SetLabelI=on  LabelI=I_Load8  Ipu=off  Pbase=100e6  Vbase=500e3  OutputType=Complex  PhasorSimulation=off  PSBequivalent=0
  BUS-Load-80 : spsThreePhaseVIMeasurementLib/Three-Phase V-I Measurement  VoltageMeasurement=phase-to-phase  SetLabelV=on  LabelV=V_Load_80  Vpu=off  VpuLL=off  CurrentMeasurement=yes  SetLabelI=on  LabelI=I_Load80  Ipu=off  Pbase=100e6  Vbase=500e3  OutputType=Complex  PhasorSimulation=off  PSBequivalent=0
  BUS-Load-81 : spsThreePhaseVIMeasurementLib/Three-Phase V-I Measurement  VoltageMeasurement=phase-to-phase  SetLabelV=on  LabelV=V_Load_81  Vpu=off  VpuLL=off  CurrentMeasurement=yes  SetLabelI=on  LabelI=I_Load81  Ipu=off  Pbase=100e6  Vbase=500e3  OutputType=Complex  PhasorSimulation=off  PSBequivalent=0
  BUS-Load-82 : spsThreePhaseVIMeasurementLib/Three-Phase V-I Measurement  VoltageMeasurement=phase-to-phase  SetLabelV=on  LabelV=V_Load_82  Vpu=off  VpuLL=off  CurrentMeasurement=yes  SetLabelI=on  LabelI=I_Load82  Ipu=off  Pbase=100e6  Vbase=500e3  OutputType=Complex  PhasorSimulation=off  PSBequivalent=0
  BUS-Load-83 : spsThreePhaseVIMeasurementLib/Three-Phase V-I Measurement  VoltageMeasurement=phase-to-phase  SetLabelV=on  LabelV=V_Load_83  Vpu=off  VpuLL=off  CurrentMeasurement=yes  SetLabelI=on  LabelI=I_Load83  Ipu=off  Pbase=100e6  Vbase=500e3  OutputType=Complex  PhasorSimulation=off  PSBequivalent=0
  BUS-Load-84 : spsThreePhaseVIMeasurementLib/Three-Phase V-I Measurement  VoltageMeasurement=phase-to-phase  SetLabelV=on  LabelV=V_Load_84  Vpu=off  VpuLL=off  CurrentMeasurement=yes  SetLabelI=on  LabelI=I_Load84  Ipu=off  Pbase=100e6  Vbase=500e3  OutputType=Complex  PhasorSimulation=off  PSBequivalent=0
  BUS-Load-85 : spsThreePhaseVIMeasurementLib/Three-Phase V-I Measurement  VoltageMeasurement=phase-to-phase  SetLabelV=on  LabelV=V_Load_85  Vpu=off  VpuLL=off  CurrentMeasurement=yes  SetLabelI=on  LabelI=I_Load85  Ipu=off  Pbase=100e6  Vbase=500e3  OutputType=Complex  PhasorSimulation=off  PSBequivalent=0
  BUS-Load-86 : spsThreePhaseVIMeasurementLib/Three-Phase V-I Measurement  VoltageMeasurement=phase-to-phase  SetLabelV=on  LabelV=V_Load_86  Vpu=off  VpuLL=off  CurrentMeasurement=yes  SetLabelI=on  LabelI=I_Load86  Ipu=off  Pbase=100e6  Vbase=500e3  OutputType=Complex  PhasorSimulation=off  PSBequivalent=0
  BUS-Load-87 : spsThreePhaseVIMeasurementLib/Three-Phase V-I Measurement  VoltageMeasurement=phase-to-phase  SetLabelV=on  LabelV=V_Load_87  Vpu=off  VpuLL=off  CurrentMeasurement=yes  SetLabelI=on  LabelI=I_Load87  Ipu=off  Pbase=100e6  Vbase=500e3  OutputType=Complex  PhasorSimulation=off  PSBequivalent=0
  BUS-Load-88 : spsThreePhaseVIMeasurementLib/Three-Phase V-I Measurement  VoltageMeasurement=phase-to-phase  SetLabelV=on  LabelV=V_Load_88  Vpu=off  VpuLL=off  CurrentMeasurement=yes  SetLabelI=on  LabelI=I_Load88  Ipu=off  Pbase=100e6  Vbase=500e3  OutputType=Complex  PhasorSimulation=off  PSBequivalent=0
  BUS-Load-89 : spsThreePhaseVIMeasurementLib/Three-Phase V-I Measurement  VoltageMeasurement=phase-to-phase  SetLabelV=on  LabelV=V_Load_89  Vpu=off  VpuLL=off  CurrentMeasurement=yes  SetLabelI=on  LabelI=I_Load89  Ipu=off  Pbase=100e6  Vbase=500e3  OutputType=Complex  PhasorSimulation=off  PSBequivalent=0
  BUS-Load-9 : spsThreePhaseVIMeasurementLib/Three-Phase V-I Measurement  VoltageMeasurement=phase-to-phase  SetLabelV=on  LabelV=V_Load_9  Vpu=off  VpuLL=off  CurrentMeasurement=yes  SetLabelI=on  LabelI=I_Load9  Ipu=off  Pbase=100e6  Vbase=500e3  OutputType=Complex  PhasorSimulation=off  PSBequivalent=0
  BUS-Load-90 : spsThreePhaseVIMeasurementLib/Three-Phase V-I Measurement  VoltageMeasurement=phase-to-phase  SetLabelV=on  LabelV=V_Load_90  Vpu=off  VpuLL=off  CurrentMeasurement=yes  SetLabelI=on  LabelI=I_Load90  Ipu=off  Pbase=100e6  Vbase=500e3  OutputType=Complex  PhasorSimulation=off  PSBequivalent=0
  BUS-Load-91 : spsThreePhaseVIMeasurementLib/Three-Phase V-I Measurement  VoltageMeasurement=phase-to-phase  SetLabelV=on  LabelV=V_Load_91  Vpu=off  VpuLL=off  CurrentMeasurement=yes  SetLabelI=on  LabelI=I_Load91  Ipu=off  Pbase=100e6  Vbase=500e3  OutputType=Complex  PhasorSimulation=off  PSBequivalent=0
  BUS-SG-1 : spsThreePhaseVIMeasurementLib/Three-Phase V-I Measurement  VoltageMeasurement=phase-to-phase  SetLabelV=on  LabelV=V_SG_1  Vpu=off  VpuLL=off  CurrentMeasurement=yes  SetLabelI=on  LabelI=I_SG1  Ipu=off  Pbase=100e6  Vbase=500e3  OutputType=Complex  PhasorSimulation=off  PSBequivalent=0
  BUS-SG-10 : spsThreePhaseVIMeasurementLib/Three-Phase V-I Measurement  VoltageMeasurement=phase-to-phase  SetLabelV=on  LabelV=V_SG_10  Vpu=off  VpuLL=off  CurrentMeasurement=yes  SetLabelI=on  LabelI=I_SG10  Ipu=off  Pbase=100e6  Vbase=500e3  OutputType=Complex  PhasorSimulation=off  PSBequivalent=0
  BUS-SG-11 : spsThreePhaseVIMeasurementLib/Three-Phase V-I Measurement  VoltageMeasurement=phase-to-phase  SetLabelV=on  LabelV=V_SG_11  Vpu=off  VpuLL=off  CurrentMeasurement=yes  SetLabelI=on  LabelI=I_SG11  Ipu=off  Pbase=100e6  Vbase=500e3  OutputType=Complex  PhasorSimulation=off  PSBequivalent=0
  BUS-SG-12 : spsThreePhaseVIMeasurementLib/Three-Phase V-I Measurement  VoltageMeasurement=phase-to-phase  SetLabelV=on  LabelV=V_SG_12  Vpu=off  VpuLL=off  CurrentMeasurement=yes  SetLabelI=on  LabelI=I_SG12  Ipu=off  Pbase=100e6  Vbase=500e3  OutputType=Complex  PhasorSimulation=off  PSBequivalent=0
  BUS-SG-13 : spsThreePhaseVIMeasurementLib/Three-Phase V-I Measurement  VoltageMeasurement=phase-to-phase  SetLabelV=on  LabelV=V_SG_13  Vpu=off  VpuLL=off  CurrentMeasurement=yes  SetLabelI=on  LabelI=I_SG13  Ipu=off  Pbase=100e6  Vbase=500e3  OutputType=Complex  PhasorSimulation=off  PSBequivalent=0
  BUS-SG-14 : spsThreePhaseVIMeasurementLib/Three-Phase V-I Measurement  VoltageMeasurement=phase-to-phase  SetLabelV=on  LabelV=V_SG_14  Vpu=off  VpuLL=off  CurrentMeasurement=yes  SetLabelI=on  LabelI=I_SG14  Ipu=off  Pbase=100e6  Vbase=500e3  OutputType=Complex  PhasorSimulation=off  PSBequivalent=0
  BUS-SG-15 : spsThreePhaseVIMeasurementLib/Three-Phase V-I Measurement  VoltageMeasurement=phase-to-phase  SetLabelV=on  LabelV=V_SG_15  Vpu=off  VpuLL=off  CurrentMeasurement=yes  SetLabelI=on  LabelI=I_SG15  Ipu=off  Pbase=100e6  Vbase=500e3  OutputType=Complex  PhasorSimulation=off  PSBequivalent=0
  BUS-SG-16 : spsThreePhaseVIMeasurementLib/Three-Phase V-I Measurement  VoltageMeasurement=phase-to-phase  SetLabelV=on  LabelV=V_SG_16  Vpu=off  VpuLL=off  CurrentMeasurement=yes  SetLabelI=on  LabelI=I_SG16  Ipu=off  Pbase=100e6  Vbase=500e3  OutputType=Complex  PhasorSimulation=off  PSBequivalent=0
  BUS-SG-17 : spsThreePhaseVIMeasurementLib/Three-Phase V-I Measurement  VoltageMeasurement=phase-to-phase  SetLabelV=on  LabelV=V_SG_17  Vpu=off  VpuLL=off  CurrentMeasurement=yes  SetLabelI=on  LabelI=I_SG17  Ipu=off  Pbase=100e6  Vbase=500e3  OutputType=Complex  PhasorSimulation=off  PSBequivalent=0
  BUS-SG-18 : spsThreePhaseVIMeasurementLib/Three-Phase V-I Measurement  VoltageMeasurement=phase-to-phase  SetLabelV=on  LabelV=V_SG_18  Vpu=off  VpuLL=off  CurrentMeasurement=yes  SetLabelI=on  LabelI=I_SG18  Ipu=off  Pbase=100e6  Vbase=500e3  OutputType=Complex  PhasorSimulation=off  PSBequivalent=0
  BUS-SG-19 : spsThreePhaseVIMeasurementLib/Three-Phase V-I Measurement  VoltageMeasurement=phase-to-phase  SetLabelV=on  LabelV=V_SG_19  Vpu=off  VpuLL=off  CurrentMeasurement=yes  SetLabelI=on  LabelI=I_SG19  Ipu=off  Pbase=100e6  Vbase=500e3  OutputType=Complex  PhasorSimulation=off  PSBequivalent=0
  BUS-SG-2 : spsThreePhaseVIMeasurementLib/Three-Phase V-I Measurement  VoltageMeasurement=phase-to-phase  SetLabelV=on  LabelV=V_SG_2  Vpu=off  VpuLL=off  CurrentMeasurement=yes  SetLabelI=on  LabelI=I_SG2  Ipu=off  Pbase=100e6  Vbase=500e3  OutputType=Complex  PhasorSimulation=off  PSBequivalent=0
  BUS-SG-20 : spsThreePhaseVIMeasurementLib/Three-Phase V-I Measurement  VoltageMeasurement=phase-to-phase  SetLabelV=on  LabelV=V_SG_20  Vpu=off  VpuLL=off  CurrentMeasurement=yes  SetLabelI=on  LabelI=I_SG20  Ipu=off  Pbase=100e6  Vbase=500e3  OutputType=Complex  PhasorSimulation=off  PSBequivalent=0
  BUS-SG-21 : spsThreePhaseVIMeasurementLib/Three-Phase V-I Measurement  VoltageMeasurement=phase-to-phase  SetLabelV=on  LabelV=V_SG_21  Vpu=off  VpuLL=off  CurrentMeasurement=yes  SetLabelI=on  LabelI=I_SG21  Ipu=off  Pbase=100e6  Vbase=500e3  OutputType=Complex  PhasorSimulation=off  PSBequivalent=0
  BUS-SG-22 : spsThreePhaseVIMeasurementLib/Three-Phase V-I Measurement  VoltageMeasurement=phase-to-phase  SetLabelV=on  LabelV=V_SG_22  Vpu=off  VpuLL=off  CurrentMeasurement=yes  SetLabelI=on  LabelI=I_SG22  Ipu=off  Pbase=100e6  Vbase=500e3  OutputType=Complex  PhasorSimulation=off  PSBequivalent=0
  BUS-SG-23 : spsThreePhaseVIMeasurementLib/Three-Phase V-I Measurement  VoltageMeasurement=phase-to-phase  SetLabelV=on  LabelV=V_SG_23  Vpu=off  VpuLL=off  CurrentMeasurement=yes  SetLabelI=on  LabelI=I_SG23  Ipu=off  Pbase=100e6  Vbase=500e3  OutputType=Complex  PhasorSimulation=off  PSBequivalent=0
  BUS-SG-24 : spsThreePhaseVIMeasurementLib/Three-Phase V-I Measurement  VoltageMeasurement=phase-to-phase  SetLabelV=on  LabelV=V_SG_24  Vpu=off  VpuLL=off  CurrentMeasurement=yes  SetLabelI=on  LabelI=I_SG24  Ipu=off  Pbase=100e6  Vbase=500e3  OutputType=Complex  PhasorSimulation=off  PSBequivalent=0
  BUS-SG-25 : spsThreePhaseVIMeasurementLib/Three-Phase V-I Measurement  VoltageMeasurement=phase-to-phase  SetLabelV=on  LabelV=V_SG_25  Vpu=off  VpuLL=off  CurrentMeasurement=yes  SetLabelI=on  LabelI=I_SG25  Ipu=off  Pbase=100e6  Vbase=500e3  OutputType=Complex  PhasorSimulation=off  PSBequivalent=0
  BUS-SG-26 : spsThreePhaseVIMeasurementLib/Three-Phase V-I Measurement  VoltageMeasurement=phase-to-phase  SetLabelV=on  LabelV=V_SG_26  Vpu=off  VpuLL=off  CurrentMeasurement=yes  SetLabelI=on  LabelI=I_SG26  Ipu=off  Pbase=100e6  Vbase=500e3  OutputType=Complex  PhasorSimulation=off  PSBequivalent=0
  BUS-SG-3 : spsThreePhaseVIMeasurementLib/Three-Phase V-I Measurement  VoltageMeasurement=phase-to-phase  SetLabelV=on  LabelV=V_SG_3  Vpu=off  VpuLL=off  CurrentMeasurement=yes  SetLabelI=on  LabelI=I_SG3  Ipu=off  Pbase=100e6  Vbase=500e3  OutputType=Complex  PhasorSimulation=off  PSBequivalent=0
  BUS-SG-4 : spsThreePhaseVIMeasurementLib/Three-Phase V-I Measurement  VoltageMeasurement=phase-to-phase  SetLabelV=on  LabelV=V_SG_4  Vpu=off  VpuLL=off  CurrentMeasurement=yes  SetLabelI=on  LabelI=I_SG4  Ipu=off  Pbase=100e6  Vbase=500e3  OutputType=Complex  PhasorSimulation=off  PSBequivalent=0
  BUS-SG-5 : spsThreePhaseVIMeasurementLib/Three-Phase V-I Measurement  VoltageMeasurement=phase-to-phase  SetLabelV=on  LabelV=V_SG_5  Vpu=off  VpuLL=off  CurrentMeasurement=yes  SetLabelI=on  LabelI=I_SG5  Ipu=off  Pbase=100e6  Vbase=500e3  OutputType=Complex  PhasorSimulation=off  PSBequivalent=0
  BUS-SG-6 : spsThreePhaseVIMeasurementLib/Three-Phase V-I Measurement  VoltageMeasurement=phase-to-phase  SetLabelV=on  LabelV=V_SG_6  Vpu=off  VpuLL=off  CurrentMeasurement=yes  SetLabelI=on  LabelI=I_SG6  Ipu=off  Pbase=100e6  Vbase=500e3  OutputType=Complex  PhasorSimulation=off  PSBequivalent=0
  BUS-SG-7 : spsThreePhaseVIMeasurementLib/Three-Phase V-I Measurement  VoltageMeasurement=phase-to-phase  SetLabelV=on  LabelV=V_SG_7  Vpu=off  VpuLL=off  CurrentMeasurement=yes  SetLabelI=on  LabelI=I_SG7  Ipu=off  Pbase=100e6  Vbase=500e3  OutputType=Complex  PhasorSimulation=off  PSBequivalent=0
  BUS-SG-8 : spsThreePhaseVIMeasurementLib/Three-Phase V-I Measurement  VoltageMeasurement=phase-to-phase  SetLabelV=on  LabelV=V_SG_8  Vpu=off  VpuLL=off  CurrentMeasurement=yes  SetLabelI=on  LabelI=I_SG8  Ipu=off  Pbase=100e6  Vbase=500e3  OutputType=Complex  PhasorSimulation=off  PSBequivalent=0
  BUS-SG-9 : spsThreePhaseVIMeasurementLib/Three-Phase V-I Measurement  VoltageMeasurement=phase-to-phase  SetLabelV=on  LabelV=V_SG_9  Vpu=off  VpuLL=off  CurrentMeasurement=yes  SetLabelI=on  LabelI=I_SG9  Ipu=off  Pbase=100e6  Vbase=500e3  OutputType=Complex  PhasorSimulation=off  PSBequivalent=0
  BUS-VSC-1 : spsThreePhaseVIMeasurementLib/Three-Phase V-I Measurement  VoltageMeasurement=phase-to-phase  SetLabelV=on  LabelV=V_VSC_1  Vpu=off  VpuLL=off  CurrentMeasurement=yes  SetLabelI=on  LabelI=I_VSC1  Ipu=off  Pbase=100e6  Vbase=500e3  OutputType=Complex  PhasorSimulation=off  PSBequivalent=0
  BUS-VSC-10 : spsThreePhaseVIMeasurementLib/Three-Phase V-I Measurement  VoltageMeasurement=phase-to-phase  SetLabelV=on  LabelV=V_VSC_10  Vpu=off  VpuLL=off  CurrentMeasurement=yes  SetLabelI=on  LabelI=I_VSC10  Ipu=off  Pbase=100e6  Vbase=500e3  OutputType=Complex  PhasorSimulation=off  PSBequivalent=0
  BUS-VSC-11 : spsThreePhaseVIMeasurementLib/Three-Phase V-I Measurement  VoltageMeasurement=phase-to-phase  SetLabelV=on  LabelV=V_VSC_11  Vpu=off  VpuLL=off  CurrentMeasurement=yes  SetLabelI=on  LabelI=I_VSC11  Ipu=off  Pbase=100e6  Vbase=500e3  OutputType=Complex  PhasorSimulation=off  PSBequivalent=0
  BUS-VSC-12 : spsThreePhaseVIMeasurementLib/Three-Phase V-I Measurement  VoltageMeasurement=phase-to-phase  SetLabelV=on  LabelV=V_VSC_12  Vpu=off  VpuLL=off  CurrentMeasurement=yes  SetLabelI=on  LabelI=I_VSC12  Ipu=off  Pbase=100e6  Vbase=500e3  OutputType=Complex  PhasorSimulation=off  PSBequivalent=0
  BUS-VSC-13 : spsThreePhaseVIMeasurementLib/Three-Phase V-I Measurement  VoltageMeasurement=phase-to-phase  SetLabelV=on  LabelV=V_VSC_13  Vpu=off  VpuLL=off  CurrentMeasurement=yes  SetLabelI=on  LabelI=I_VSC13  Ipu=off  Pbase=100e6  Vbase=500e3  OutputType=Complex  PhasorSimulation=off  PSBequivalent=0
  BUS-VSC-14 : spsThreePhaseVIMeasurementLib/Three-Phase V-I Measurement  VoltageMeasurement=phase-to-phase  SetLabelV=on  LabelV=V_VSC_14  Vpu=off  VpuLL=off  CurrentMeasurement=yes  SetLabelI=on  LabelI=I_VSC14  Ipu=off  Pbase=100e6  Vbase=500e3  OutputType=Complex  PhasorSimulation=off  PSBequivalent=0
  BUS-VSC-15 : spsThreePhaseVIMeasurementLib/Three-Phase V-I Measurement  VoltageMeasurement=phase-to-phase  SetLabelV=on  LabelV=V_VSC_15  Vpu=off  VpuLL=off  CurrentMeasurement=yes  SetLabelI=on  LabelI=I_VSC15  Ipu=off  Pbase=100e6  Vbase=500e3  OutputType=Complex  PhasorSimulation=off  PSBequivalent=0
  BUS-VSC-16 : spsThreePhaseVIMeasurementLib/Three-Phase V-I Measurement  VoltageMeasurement=phase-to-phase  SetLabelV=on  LabelV=V_VSC_16  Vpu=off  VpuLL=off  CurrentMeasurement=yes  SetLabelI=on  LabelI=I_VSC16  Ipu=off  Pbase=100e6  Vbase=500e3  OutputType=Complex  PhasorSimulation=off  PSBequivalent=0
  BUS-VSC-17 : spsThreePhaseVIMeasurementLib/Three-Phase V-I Measurement  VoltageMeasurement=phase-to-phase  SetLabelV=on  LabelV=V_VSC_17  Vpu=off  VpuLL=off  CurrentMeasurement=yes  SetLabelI=on  LabelI=I_VSC17  Ipu=off  Pbase=100e6  Vbase=500e3  OutputType=Complex  PhasorSimulation=off  PSBequivalent=0
  BUS-VSC-18 : spsThreePhaseVIMeasurementLib/Three-Phase V-I Measurement  VoltageMeasurement=phase-to-phase  SetLabelV=on  LabelV=V_VSC_18  Vpu=off  VpuLL=off  CurrentMeasurement=yes  SetLabelI=on  LabelI=I_VSC18  Ipu=off  Pbase=100e6  Vbase=500e3  OutputType=Complex  PhasorSimulation=off  PSBequivalent=0
  BUS-VSC-19 : spsThreePhaseVIMeasurementLib/Three-Phase V-I Measurement  VoltageMeasurement=phase-to-phase  SetLabelV=on  LabelV=V_VSC_19  Vpu=off  VpuLL=off  CurrentMeasurement=yes  SetLabelI=on  LabelI=I_VSC19  Ipu=off  Pbase=100e6  Vbase=500e3  OutputType=Complex  PhasorSimulation=off  PSBequivalent=0
  BUS-VSC-2 : spsThreePhaseVIMeasurementLib/Three-Phase V-I Measurement  VoltageMeasurement=phase-to-phase  SetLabelV=on  LabelV=V_VSC_2  Vpu=off  VpuLL=off  CurrentMeasurement=yes  SetLabelI=on  LabelI=I_VSC2  Ipu=off  Pbase=100e6  Vbase=500e3  OutputType=Complex  PhasorSimulation=off  PSBequivalent=0
  BUS-VSC-20 : spsThreePhaseVIMeasurementLib/Three-Phase V-I Measurement  VoltageMeasurement=phase-to-phase  SetLabelV=on  LabelV=V_VSC_20  Vpu=off  VpuLL=off  CurrentMeasurement=yes  SetLabelI=on  LabelI=I_VSC20  Ipu=off  Pbase=100e6  Vbase=500e3  OutputType=Complex  PhasorSimulation=off  PSBequivalent=0
  BUS-VSC-3 : spsThreePhaseVIMeasurementLib/Three-Phase V-I Measurement  VoltageMeasurement=phase-to-phase  SetLabelV=on  LabelV=V_VSC_3  Vpu=off  VpuLL=off  CurrentMeasurement=yes  SetLabelI=on  LabelI=I_VSC3  Ipu=off  Pbase=100e6  Vbase=500e3  OutputType=Complex  PhasorSimulation=off  PSBequivalent=0
  BUS-VSC-4 : spsThreePhaseVIMeasurementLib/Three-Phase V-I Measurement  VoltageMeasurement=phase-to-phase  SetLabelV=on  LabelV=V_VSC_4  Vpu=off  VpuLL=off  CurrentMeasurement=yes  SetLabelI=on  LabelI=I_VSC4  Ipu=off  Pbase=100e6  Vbase=500e3  OutputType=Complex  PhasorSimulation=off  PSBequivalent=0
  BUS-VSC-5 : spsThreePhaseVIMeasurementLib/Three-Phase V-I Measurement  VoltageMeasurement=phase-to-phase  SetLabelV=on  LabelV=V_VSC_5  Vpu=off  VpuLL=off  CurrentMeasurement=yes  SetLabelI=on  LabelI=I_VSC5  Ipu=off  Pbase=100e6  Vbase=500e3  OutputType=Complex  PhasorSimulation=off  PSBequivalent=0
  BUS-VSC-6 : spsThreePhaseVIMeasurementLib/Three-Phase V-I Measurement  VoltageMeasurement=phase-to-phase  SetLabelV=on  LabelV=V_VSC_6  Vpu=off  VpuLL=off  CurrentMeasurement=yes  SetLabelI=on  LabelI=I_VSC6  Ipu=off  Pbase=100e6  Vbase=500e3  OutputType=Complex  PhasorSimulation=off  PSBequivalent=0
  BUS-VSC-7 : spsThreePhaseVIMeasurementLib/Three-Phase V-I Measurement  VoltageMeasurement=phase-to-phase  SetLabelV=on  LabelV=V_VSC_7  Vpu=off  VpuLL=off  CurrentMeasurement=yes  SetLabelI=on  LabelI=I_VSC7  Ipu=off  Pbase=100e6  Vbase=500e3  OutputType=Complex  PhasorSimulation=off  PSBequivalent=0
  BUS-VSC-8 : spsThreePhaseVIMeasurementLib/Three-Phase V-I Measurement  VoltageMeasurement=phase-to-phase  SetLabelV=on  LabelV=V_VSC_8  Vpu=off  VpuLL=off  CurrentMeasurement=yes  SetLabelI=on  LabelI=I_VSC8  Ipu=off  Pbase=100e6  Vbase=500e3  OutputType=Complex  PhasorSimulation=off  PSBequivalent=0
  BUS-VSC-9 : spsThreePhaseVIMeasurementLib/Three-Phase V-I Measurement  VoltageMeasurement=phase-to-phase  SetLabelV=on  LabelV=V_VSC_9  Vpu=off  VpuLL=off  CurrentMeasurement=yes  SetLabelI=on  LabelI=I_VSC9  Ipu=off  Pbase=100e6  Vbase=500e3  OutputType=Complex  PhasorSimulation=off  PSBequivalent=0
  Constant{,1..112} (113 alike) : Constant  Value=[2/3 1/3; -1/3 1/3 ; -1/3 -2/3]
  Demux{,1..112} (113 alike) : Demux  Outputs=3
  Line-1 : myLibrary/PI_line  T_line_global=T_NET  initLine_global=init_line  num=1  set_C0=ones(1,6)  set_iL0=0
  Line-10 : myLibrary/PI_line  T_line_global=T_NET  initLine_global=init_line  num=10  set_C0=ones(1,6)  set_iL0=0
  Line-100 : myLibrary/PI_line  T_line_global=T_NET  initLine_global=init_line  num=100  set_C0=ones(1,6)  set_iL0=0
  Line-101 : myLibrary/PI_line  T_line_global=T_NET  initLine_global=init_line  num=101  set_C0=ones(1,6)  set_iL0=0
  Line-102 : myLibrary/PI_line  T_line_global=T_NET  initLine_global=init_line  num=102  set_C0=ones(1,6)  set_iL0=0
  Line-103 : myLibrary/PI_line  T_line_global=T_NET  initLine_global=init_line  num=103  set_C0=ones(1,6)  set_iL0=0
  Line-104 : myLibrary/PI_line  T_line_global=T_NET  initLine_global=init_line  num=104  set_C0=ones(1,6)  set_iL0=0
  Line-105 : myLibrary/PI_line  T_line_global=T_NET  initLine_global=init_line  num=105  set_C0=ones(1,6)  set_iL0=0
  Line-106 : myLibrary/PI_line  T_line_global=T_NET  initLine_global=init_line  num=106  set_C0=ones(1,6)  set_iL0=0
  Line-107 : myLibrary/PI_line  T_line_global=T_NET  initLine_global=init_line  num=107  set_C0=ones(1,6)  set_iL0=0
  Line-108 : myLibrary/PI_line  T_line_global=T_NET  initLine_global=init_line  num=108  set_C0=ones(1,6)  set_iL0=0
  Line-109 : myLibrary/PI_line  T_line_global=T_NET  initLine_global=init_line  num=109  set_C0=ones(1,6)  set_iL0=0
  Line-11 : myLibrary/PI_line  T_line_global=T_NET  initLine_global=init_line  num=11  set_C0=ones(1,6)  set_iL0=0
  Line-110 : myLibrary/PI_line  T_line_global=T_NET  initLine_global=init_line  num=110  set_C0=ones(1,6)  set_iL0=0
  Line-111 : myLibrary/PI_line  T_line_global=T_NET  initLine_global=init_line  num=111  set_C0=ones(1,6)  set_iL0=0
  Line-112 : myLibrary/PI_line  T_line_global=T_NET  initLine_global=init_line  num=112  set_C0=ones(1,6)  set_iL0=0
  Line-113 : myLibrary/PI_line  T_line_global=T_NET  initLine_global=init_line  num=113  set_C0=ones(1,6)  set_iL0=0
  Line-114 : myLibrary/PI_line  T_line_global=T_NET  initLine_global=init_line  num=114  set_C0=ones(1,6)  set_iL0=0
  Line-115 : myLibrary/PI_line  T_line_global=T_NET  initLine_global=init_line  num=115  set_C0=ones(1,6)  set_iL0=0
  Line-116 : myLibrary/PI_line  T_line_global=T_NET  initLine_global=init_line  num=116  set_C0=ones(1,6)  set_iL0=0
  Line-117 : myLibrary/PI_line  T_line_global=T_NET  initLine_global=init_line  num=117  set_C0=ones(1,6)  set_iL0=0
  Line-118 : myLibrary/PI_line  T_line_global=T_NET  initLine_global=init_line  num=118  set_C0=ones(1,6)  set_iL0=0
  Line-119 : myLibrary/PI_line  T_line_global=T_NET  initLine_global=init_line  num=119  set_C0=ones(1,6)  set_iL0=0
  Line-12 : myLibrary/PI_line  T_line_global=T_NET  initLine_global=init_line  num=12  set_C0=ones(1,6)  set_iL0=0
  Line-120 : myLibrary/PI_line  T_line_global=T_NET  initLine_global=init_line  num=120  set_C0=ones(1,6)  set_iL0=0
  Line-121 : myLibrary/PI_line  T_line_global=T_NET  initLine_global=init_line  num=121  set_C0=ones(1,6)  set_iL0=0
  Line-122 : myLibrary/PI_line  T_line_global=T_NET  initLine_global=init_line  num=122  set_C0=ones(1,6)  set_iL0=0
  Line-123 : myLibrary/PI_line  T_line_global=T_NET  initLine_global=init_line  num=123  set_C0=ones(1,6)  set_iL0=0
  Line-124 : myLibrary/PI_line  T_line_global=T_NET  initLine_global=init_line  num=124  set_C0=ones(1,6)  set_iL0=0
  Line-125 : myLibrary/PI_line  T_line_global=T_NET  initLine_global=init_line  num=125  set_C0=ones(1,6)  set_iL0=0
  Line-126 : myLibrary/PI_line  T_line_global=T_NET  initLine_global=init_line  num=126  set_C0=ones(1,6)  set_iL0=0
  Line-127 : myLibrary/PI_line  T_line_global=T_NET  initLine_global=init_line  num=127  set_C0=ones(1,6)  set_iL0=0
  Line-128 : myLibrary/PI_line  T_line_global=T_NET  initLine_global=init_line  num=128  set_C0=ones(1,6)  set_iL0=0
  Line-129 : myLibrary/PI_line  T_line_global=T_NET  initLine_global=init_line  num=129  set_C0=ones(1,6)  set_iL0=0
  Line-13 : myLibrary/PI_line  T_line_global=T_NET  initLine_global=init_line  num=13  set_C0=ones(1,6)  set_iL0=0
  Line-130 : myLibrary/PI_line  T_line_global=T_NET  initLine_global=init_line  num=130  set_C0=ones(1,6)  set_iL0=0
  Line-131 : myLibrary/PI_line  T_line_global=T_NET  initLine_global=init_line  num=131  set_C0=ones(1,6)  set_iL0=0
  Line-132 : myLibrary/PI_line  T_line_global=T_NET  initLine_global=init_line  num=132  set_C0=ones(1,6)  set_iL0=0
  Line-133 : myLibrary/PI_line  T_line_global=T_NET  initLine_global=init_line  num=133  set_C0=ones(1,6)  set_iL0=0
  Line-134 : myLibrary/PI_line  T_line_global=T_NET  initLine_global=init_line  num=134  set_C0=ones(1,6)  set_iL0=0
  Line-135 : myLibrary/PI_line  T_line_global=T_NET  initLine_global=init_line  num=135  set_C0=ones(1,6)  set_iL0=0
  Line-136 : myLibrary/PI_line  T_line_global=T_NET  initLine_global=init_line  num=136  set_C0=ones(1,6)  set_iL0=0
  Line-137 : myLibrary/PI_line  T_line_global=T_NET  initLine_global=init_line  num=137  set_C0=ones(1,6)  set_iL0=0
  Line-138 : myLibrary/PI_line  T_line_global=T_NET  initLine_global=init_line  num=138  set_C0=ones(1,6)  set_iL0=0
  Line-139 : myLibrary/PI_line  T_line_global=T_NET  initLine_global=init_line  num=139  set_C0=ones(1,6)  set_iL0=0
  Line-14 : myLibrary/PI_line  T_line_global=T_NET  initLine_global=init_line  num=14  set_C0=ones(1,6)  set_iL0=0
  Line-140 : myLibrary/PI_line  T_line_global=T_NET  initLine_global=init_line  num=140  set_C0=ones(1,6)  set_iL0=0
  Line-141 : myLibrary/PI_line  T_line_global=T_NET  initLine_global=init_line  num=141  set_C0=ones(1,6)  set_iL0=0
  Line-142 : myLibrary/PI_line  T_line_global=T_NET  initLine_global=init_line  num=142  set_C0=ones(1,6)  set_iL0=0
  Line-143 : myLibrary/PI_line  T_line_global=T_NET  initLine_global=init_line  num=143  set_C0=ones(1,6)  set_iL0=0
  Line-144 : myLibrary/PI_line  T_line_global=T_NET  initLine_global=init_line  num=144  set_C0=ones(1,6)  set_iL0=0
  Line-145 : myLibrary/PI_line  T_line_global=T_NET  initLine_global=init_line  num=145  set_C0=ones(1,6)  set_iL0=0
  Line-146 : myLibrary/PI_line  T_line_global=T_NET  initLine_global=init_line  num=146  set_C0=ones(1,6)  set_iL0=0
  Line-147 : myLibrary/PI_line  T_line_global=T_NET  initLine_global=init_line  num=147  set_C0=ones(1,6)  set_iL0=0
  Line-148 : myLibrary/PI_line  T_line_global=T_NET  initLine_global=init_line  num=148  set_C0=ones(1,6)  set_iL0=0
  Line-149 : myLibrary/PI_line  T_line_global=T_NET  initLine_global=init_line  num=149  set_C0=ones(1,6)  set_iL0=0
  Line-15 : myLibrary/PI_line  T_line_global=T_NET  initLine_global=init_line  num=15  set_C0=ones(1,6)  set_iL0=0
  Line-150 : myLibrary/PI_line  T_line_global=T_NET  initLine_global=init_line  num=150  set_C0=ones(1,6)  set_iL0=0
  Line-151 : myLibrary/PI_line  T_line_global=T_NET  initLine_global=init_line  num=151  set_C0=ones(1,6)  set_iL0=0
  Line-152 : myLibrary/PI_line  T_line_global=T_NET  initLine_global=init_line  num=152  set_C0=ones(1,6)  set_iL0=0
  Line-153 : myLibrary/PI_line  T_line_global=T_NET  initLine_global=init_line  num=153  set_C0=ones(1,6)  set_iL0=0
  Line-154 : myLibrary/PI_line  T_line_global=T_NET  initLine_global=init_line  num=154  set_C0=ones(1,6)  set_iL0=0
  Line-155 : myLibrary/PI_line  T_line_global=T_NET  initLine_global=init_line  num=155  set_C0=ones(1,6)  set_iL0=0
  Line-156 : myLibrary/PI_line  T_line_global=T_NET  initLine_global=init_line  num=156  set_C0=ones(1,6)  set_iL0=0
  Line-157 : myLibrary/PI_line  T_line_global=T_NET  initLine_global=init_line  num=157  set_C0=ones(1,6)  set_iL0=0
  Line-158 : myLibrary/PI_line  T_line_global=T_NET  initLine_global=init_line  num=158  set_C0=ones(1,6)  set_iL0=0
  Line-159 : myLibrary/PI_line  T_line_global=T_NET  initLine_global=init_line  num=159  set_C0=ones(1,6)  set_iL0=0
  Line-16 : myLibrary/PI_line  T_line_global=T_NET  initLine_global=init_line  num=16  set_C0=ones(1,6)  set_iL0=0
  Line-160 : myLibrary/PI_line  T_line_global=T_NET  initLine_global=init_line  num=160  set_C0=ones(1,6)  set_iL0=0
  Line-161 : myLibrary/PI_line  T_line_global=T_NET  initLine_global=init_line  num=161  set_C0=ones(1,6)  set_iL0=0
  Line-162 : myLibrary/PI_line  T_line_global=T_NET  initLine_global=init_line  num=162  set_C0=ones(1,6)  set_iL0=0
  Line-163 : myLibrary/PI_line  T_line_global=T_NET  initLine_global=init_line  num=163  set_C0=ones(1,6)  set_iL0=0
  Line-164 : myLibrary/PI_line  T_line_global=T_NET  initLine_global=init_line  num=164  set_C0=ones(1,6)  set_iL0=0
  Line-165 : myLibrary/PI_line  T_line_global=T_NET  initLine_global=init_line  num=165  set_C0=ones(1,6)  set_iL0=0
  Line-166 : myLibrary/RL_line  T_line_global=T_NET  initLine_global=init_line  num=166
  Line-167 : myLibrary/RL_line  T_line_global=T_NET  initLine_global=init_line  num=167
  Line-168 : myLibrary/RL_line  T_line_global=T_NET  initLine_global=init_line  num=168
  Line-169 : myLibrary/RL_line  T_line_global=T_NET  initLine_global=init_line  num=169
  Line-17 : myLibrary/PI_line  T_line_global=T_NET  initLine_global=init_line  num=17  set_C0=ones(1,6)  set_iL0=0
  Line-170 : myLibrary/RL_line  T_line_global=T_NET  initLine_global=init_line  num=170
  Line-171 : myLibrary/RL_line  T_line_global=T_NET  initLine_global=init_line  num=171
  Line-172 : myLibrary/RL_line  T_line_global=T_NET  initLine_global=init_line  num=172
  Line-173 : myLibrary/RL_line  T_line_global=T_NET  initLine_global=init_line  num=173
  Line-174 : myLibrary/RL_line  T_line_global=T_NET  initLine_global=init_line  num=174
  Line-18 : myLibrary/PI_line  T_line_global=T_NET  initLine_global=init_line  num=18  set_C0=ones(1,6)  set_iL0=0
  Line-19 : myLibrary/PI_line  T_line_global=T_NET  initLine_global=init_line  num=19  set_C0=ones(1,6)  set_iL0=0
  Line-2 : myLibrary/PI_line  T_line_global=T_NET  initLine_global=init_line  num=2  set_C0=ones(1,6)  set_iL0=0
  Line-20 : myLibrary/PI_line  T_line_global=T_NET  initLine_global=init_line  num=20  set_C0=ones(1,6)  set_iL0=0
  Line-21 : myLibrary/PI_line  T_line_global=T_NET  initLine_global=init_line  num=21  set_C0=ones(1,6)  set_iL0=0
  Line-22 : myLibrary/PI_line  T_line_global=T_NET  initLine_global=init_line  num=22  set_C0=ones(1,6)  set_iL0=0
  Line-23 : myLibrary/PI_line  T_line_global=T_NET  initLine_global=init_line  num=23  set_C0=ones(1,6)  set_iL0=0
  Line-24 : myLibrary/PI_line  T_line_global=T_NET  initLine_global=init_line  num=24  set_C0=ones(1,6)  set_iL0=0
  Line-25 : myLibrary/PI_line  T_line_global=T_NET  initLine_global=init_line  num=25  set_C0=ones(1,6)  set_iL0=0
  Line-26 : myLibrary/PI_line  T_line_global=T_NET  initLine_global=init_line  num=26  set_C0=ones(1,6)  set_iL0=0
  Line-27 : myLibrary/PI_line  T_line_global=T_NET  initLine_global=init_line  num=27  set_C0=ones(1,6)  set_iL0=0
  Line-28 : myLibrary/PI_line  T_line_global=T_NET  initLine_global=init_line  num=28  set_C0=ones(1,6)  set_iL0=0
  Line-29 : myLibrary/PI_line  T_line_global=T_NET  initLine_global=init_line  num=29  set_C0=ones(1,6)  set_iL0=0
  Line-3 : myLibrary/PI_line  T_line_global=T_NET  initLine_global=init_line  num=3  set_C0=ones(1,6)  set_iL0=0
  Line-30 : myLibrary/PI_line  T_line_global=T_NET  initLine_global=init_line  num=30  set_C0=ones(1,6)  set_iL0=0
  Line-31 : myLibrary/PI_line  T_line_global=T_NET  initLine_global=init_line  num=31  set_C0=ones(1,6)  set_iL0=0
  Line-32 : myLibrary/PI_line  T_line_global=T_NET  initLine_global=init_line  num=32  set_C0=ones(1,6)  set_iL0=0
  Line-33 : myLibrary/PI_line  T_line_global=T_NET  initLine_global=init_line  num=33  set_C0=ones(1,6)  set_iL0=0
  Line-34 : myLibrary/PI_line  T_line_global=T_NET  initLine_global=init_line  num=34  set_C0=ones(1,6)  set_iL0=0
  Line-35 : myLibrary/PI_line  T_line_global=T_NET  initLine_global=init_line  num=35  set_C0=ones(1,6)  set_iL0=0
  Line-36 : myLibrary/PI_line  T_line_global=T_NET  initLine_global=init_line  num=36  set_C0=ones(1,6)  set_iL0=0
  Line-37 : myLibrary/PI_line  T_line_global=T_NET  initLine_global=init_line  num=37  set_C0=ones(1,6)  set_iL0=0
  Line-38 : myLibrary/PI_line  T_line_global=T_NET  initLine_global=init_line  num=38  set_C0=ones(1,6)  set_iL0=0
  Line-39 : myLibrary/PI_line  T_line_global=T_NET  initLine_global=init_line  num=39  set_C0=ones(1,6)  set_iL0=0
  Line-4 : myLibrary/PI_line  T_line_global=T_NET  initLine_global=init_line  num=4  set_C0=ones(1,6)  set_iL0=0
  Line-40 : myLibrary/PI_line  T_line_global=T_NET  initLine_global=init_line  num=40  set_C0=ones(1,6)  set_iL0=0
  Line-41 : myLibrary/PI_line  T_line_global=T_NET  initLine_global=init_line  num=41  set_C0=ones(1,6)  set_iL0=0
  Line-42 : myLibrary/PI_line  T_line_global=T_NET  initLine_global=init_line  num=42  set_C0=ones(1,6)  set_iL0=0
  Line-43 : myLibrary/PI_line  T_line_global=T_NET  initLine_global=init_line  num=43  set_C0=ones(1,6)  set_iL0=0
  Line-44 : myLibrary/PI_line  T_line_global=T_NET  initLine_global=init_line  num=44  set_C0=ones(1,6)  set_iL0=0
  Line-45 : myLibrary/PI_line  T_line_global=T_NET  initLine_global=init_line  num=45  set_C0=ones(1,6)  set_iL0=0
  Line-46 : myLibrary/PI_line  T_line_global=T_NET  initLine_global=init_line  num=46  set_C0=ones(1,6)  set_iL0=0
  Line-47 : myLibrary/PI_line  T_line_global=T_NET  initLine_global=init_line  num=47  set_C0=ones(1,6)  set_iL0=0
  Line-48 : myLibrary/PI_line  T_line_global=T_NET  initLine_global=init_line  num=48  set_C0=ones(1,6)  set_iL0=0
  Line-49 : myLibrary/PI_line  T_line_global=T_NET  initLine_global=init_line  num=49  set_C0=ones(1,6)  set_iL0=0
  Line-5 : myLibrary/PI_line  T_line_global=T_NET  initLine_global=init_line  num=5  set_C0=ones(1,6)  set_iL0=0
  Line-50 : myLibrary/PI_line  T_line_global=T_NET  initLine_global=init_line  num=50  set_C0=ones(1,6)  set_iL0=0
  Line-51 : myLibrary/PI_line  T_line_global=T_NET  initLine_global=init_line  num=51  set_C0=ones(1,6)  set_iL0=0
  Line-52 : myLibrary/PI_line  T_line_global=T_NET  initLine_global=init_line  num=52  set_C0=ones(1,6)  set_iL0=0
  Line-53 : myLibrary/PI_line  T_line_global=T_NET  initLine_global=init_line  num=53  set_C0=ones(1,6)  set_iL0=0
  Line-54 : myLibrary/PI_line  T_line_global=T_NET  initLine_global=init_line  num=54  set_C0=ones(1,6)  set_iL0=0
  Line-55 : myLibrary/PI_line  T_line_global=T_NET  initLine_global=init_line  num=55  set_C0=ones(1,6)  set_iL0=0
  Line-56 : myLibrary/PI_line  T_line_global=T_NET  initLine_global=init_line  num=56  set_C0=ones(1,6)  set_iL0=0
  Line-57 : myLibrary/PI_line  T_line_global=T_NET  initLine_global=init_line  num=57  set_C0=ones(1,6)  set_iL0=0
  Line-58 : myLibrary/PI_line  T_line_global=T_NET  initLine_global=init_line  num=58  set_C0=ones(1,6)  set_iL0=0
  Line-59 : myLibrary/PI_line  T_line_global=T_NET  initLine_global=init_line  num=59  set_C0=ones(1,6)  set_iL0=0
  Line-6 : myLibrary/PI_line  T_line_global=T_NET  initLine_global=init_line  num=6  set_C0=ones(1,6)  set_iL0=0
  Line-60 : myLibrary/PI_line  T_line_global=T_NET  initLine_global=init_line  num=60  set_C0=ones(1,6)  set_iL0=0
  Line-61 : myLibrary/PI_line  T_line_global=T_NET  initLine_global=init_line  num=61  set_C0=ones(1,6)  set_iL0=0
  Line-62 : myLibrary/PI_line  T_line_global=T_NET  initLine_global=init_line  num=62  set_C0=ones(1,6)  set_iL0=0
  Line-63 : myLibrary/PI_line  T_line_global=T_NET  initLine_global=init_line  num=63  set_C0=ones(1,6)  set_iL0=0
  Line-64 : myLibrary/PI_line  T_line_global=T_NET  initLine_global=init_line  num=64  set_C0=ones(1,6)  set_iL0=0
  Line-65 : myLibrary/PI_line  T_line_global=T_NET  initLine_global=init_line  num=65  set_C0=ones(1,6)  set_iL0=0
  Line-66 : myLibrary/PI_line  T_line_global=T_NET  initLine_global=init_line  num=66  set_C0=ones(1,6)  set_iL0=0
  Line-67 : myLibrary/PI_line  T_line_global=T_NET  initLine_global=init_line  num=67  set_C0=ones(1,6)  set_iL0=0
  Line-68 : myLibrary/PI_line  T_line_global=T_NET  initLine_global=init_line  num=68  set_C0=ones(1,6)  set_iL0=0
  Line-69 : myLibrary/PI_line  T_line_global=T_NET  initLine_global=init_line  num=69  set_C0=ones(1,6)  set_iL0=0
  Line-7 : myLibrary/PI_line  T_line_global=T_NET  initLine_global=init_line  num=7  set_C0=ones(1,6)  set_iL0=0
  Line-70 : myLibrary/PI_line  T_line_global=T_NET  initLine_global=init_line  num=70  set_C0=ones(1,6)  set_iL0=0
  Line-71 : myLibrary/PI_line  T_line_global=T_NET  initLine_global=init_line  num=71  set_C0=ones(1,6)  set_iL0=0
  Line-72 : myLibrary/PI_line  T_line_global=T_NET  initLine_global=init_line  num=72  set_C0=ones(1,6)  set_iL0=0
  Line-73 : myLibrary/PI_line  T_line_global=T_NET  initLine_global=init_line  num=73  set_C0=ones(1,6)  set_iL0=0
  Line-74 : myLibrary/PI_line  T_line_global=T_NET  initLine_global=init_line  num=74  set_C0=ones(1,6)  set_iL0=0
  Line-75 : myLibrary/PI_line  T_line_global=T_NET  initLine_global=init_line  num=75  set_C0=ones(1,6)  set_iL0=0
  Line-76 : myLibrary/PI_line  T_line_global=T_NET  initLine_global=init_line  num=76  set_C0=ones(1,6)  set_iL0=0
  Line-77 : myLibrary/PI_line  T_line_global=T_NET  initLine_global=init_line  num=77  set_C0=ones(1,6)  set_iL0=0
  Line-78 : myLibrary/PI_line  T_line_global=T_NET  initLine_global=init_line  num=78  set_C0=ones(1,6)  set_iL0=0
  Line-79 : myLibrary/PI_line  T_line_global=T_NET  initLine_global=init_line  num=79  set_C0=ones(1,6)  set_iL0=0
  Line-8 : myLibrary/PI_line  T_line_global=T_NET  initLine_global=init_line  num=8  set_C0=ones(1,6)  set_iL0=0
  Line-80 : myLibrary/PI_line  T_line_global=T_NET  initLine_global=init_line  num=80  set_C0=ones(1,6)  set_iL0=0
  Line-81 : myLibrary/PI_line  T_line_global=T_NET  initLine_global=init_line  num=81  set_C0=ones(1,6)  set_iL0=0
  Line-82 : myLibrary/PI_line  T_line_global=T_NET  initLine_global=init_line  num=82  set_C0=ones(1,6)  set_iL0=0
  Line-83 : myLibrary/PI_line  T_line_global=T_NET  initLine_global=init_line  num=83  set_C0=ones(1,6)  set_iL0=0
  Line-84 : myLibrary/PI_line  T_line_global=T_NET  initLine_global=init_line  num=84  set_C0=ones(1,6)  set_iL0=0
  Line-85 : myLibrary/PI_line  T_line_global=T_NET  initLine_global=init_line  num=85  set_C0=ones(1,6)  set_iL0=0
  Line-86 : myLibrary/PI_line  T_line_global=T_NET  initLine_global=init_line  num=86  set_C0=ones(1,6)  set_iL0=0
  Line-87 : myLibrary/PI_line  T_line_global=T_NET  initLine_global=init_line  num=87  set_C0=ones(1,6)  set_iL0=0
  Line-88 : myLibrary/PI_line  T_line_global=T_NET  initLine_global=init_line  num=88  set_C0=ones(1,6)  set_iL0=0
  Line-89 : myLibrary/PI_line  T_line_global=T_NET  initLine_global=init_line  num=89  set_C0=ones(1,6)  set_iL0=0
  Line-9 : myLibrary/PI_line  T_line_global=T_NET  initLine_global=init_line  num=9  set_C0=ones(1,6)  set_iL0=0
  Line-90 : myLibrary/PI_line  T_line_global=T_NET  initLine_global=init_line  num=90  set_C0=ones(1,6)  set_iL0=0
  Line-91 : myLibrary/PI_line  T_line_global=T_NET  initLine_global=init_line  num=91  set_C0=ones(1,6)  set_iL0=0
  Line-92 : myLibrary/PI_line  T_line_global=T_NET  initLine_global=init_line  num=92  set_C0=ones(1,6)  set_iL0=0
  Line-93 : myLibrary/PI_line  T_line_global=T_NET  initLine_global=init_line  num=93  set_C0=ones(1,6)  set_iL0=0
  Line-94 : myLibrary/PI_line  T_line_global=T_NET  initLine_global=init_line  num=94  set_C0=ones(1,6)  set_iL0=0
  Line-95 : myLibrary/PI_line  T_line_global=T_NET  initLine_global=init_line  num=95  set_C0=ones(1,6)  set_iL0=0
  Line-96 : myLibrary/PI_line  T_line_global=T_NET  initLine_global=init_line  num=96  set_C0=ones(1,6)  set_iL0=0
  Line-97 : myLibrary/PI_line  T_line_global=T_NET  initLine_global=init_line  num=97  set_C0=ones(1,6)  set_iL0=0
  Line-98 : myLibrary/PI_line  T_line_global=T_NET  initLine_global=init_line  num=98  set_C0=ones(1,6)  set_iL0=0
  Line-99 : myLibrary/PI_line  T_line_global=T_NET  initLine_global=init_line  num=99  set_C0=ones(1,6)  set_iL0=0
  Load-1 : myLibrary/Load  T_load_global=T_load  initLoad_global=init_load  num=1
  Load-10 : myLibrary/Load  T_load_global=T_load  initLoad_global=init_load  num=10
  Load-11 : myLibrary/Load  T_load_global=T_load  initLoad_global=init_load  num=11
  Load-12 : myLibrary/Load  T_load_global=T_load  initLoad_global=init_load  num=12
  Load-13 : myLibrary/Load  T_load_global=T_load  initLoad_global=init_load  num=13
  Load-14 : myLibrary/Load  T_load_global=T_load  initLoad_global=init_load  num=14
  Load-15 : myLibrary/Load  T_load_global=T_load  initLoad_global=init_load  num=15
  Load-16 : myLibrary/Load  T_load_global=T_load  initLoad_global=init_load  num=16
  Load-17 : myLibrary/Load  T_load_global=T_load  initLoad_global=init_load  num=17
  Load-18 : myLibrary/Load  T_load_global=T_load  initLoad_global=init_load  num=18
  Load-19 : myLibrary/Load  T_load_global=T_load  initLoad_global=init_load  num=19
  Load-2 : myLibrary/Load  T_load_global=T_load  initLoad_global=init_load  num=2
  Load-20 : myLibrary/Load  T_load_global=T_load  initLoad_global=init_load  num=20
  Load-21 : myLibrary/Load  T_load_global=T_load  initLoad_global=init_load  num=21
  Load-22 : myLibrary/Load  T_load_global=T_load  initLoad_global=init_load  num=22
  Load-23 : myLibrary/Load  T_load_global=T_load  initLoad_global=init_load  num=23
  Load-24 : myLibrary/Load  T_load_global=T_load  initLoad_global=init_load  num=24
  Load-25 : myLibrary/Load  T_load_global=T_load  initLoad_global=init_load  num=25
  Load-26 : myLibrary/Load  T_load_global=T_load  initLoad_global=init_load  num=26
  Load-27 : myLibrary/Load  T_load_global=T_load  initLoad_global=init_load  num=27
  Load-28 : myLibrary/Load  T_load_global=T_load  initLoad_global=init_load  num=28
  Load-29 : myLibrary/Load  T_load_global=T_load  initLoad_global=init_load  num=29
  Load-3 : myLibrary/Load  T_load_global=T_load  initLoad_global=init_load  num=3
  Load-30 : myLibrary/Load  T_load_global=T_load  initLoad_global=init_load  num=30
  Load-31 : myLibrary/Load  T_load_global=T_load  initLoad_global=init_load  num=31
  Load-32 : myLibrary/Load  T_load_global=T_load  initLoad_global=init_load  num=32
  Load-33 : myLibrary/Load  T_load_global=T_load  initLoad_global=init_load  num=33
  Load-34 : myLibrary/Load  T_load_global=T_load  initLoad_global=init_load  num=34
  Load-35 : myLibrary/Load  T_load_global=T_load  initLoad_global=init_load  num=35
  Load-36 : myLibrary/Load  T_load_global=T_load  initLoad_global=init_load  num=36
  Load-37 : myLibrary/Load  T_load_global=T_load  initLoad_global=init_load  num=37
  Load-38 : myLibrary/Load  T_load_global=T_load  initLoad_global=init_load  num=38
  Load-39 : myLibrary/Load  T_load_global=T_load  initLoad_global=init_load  num=39
  Load-4 : myLibrary/Load  T_load_global=T_load  initLoad_global=init_load  num=4
  Load-40 : myLibrary/Load  T_load_global=T_load  initLoad_global=init_load  num=40
  Load-41 : myLibrary/Load  T_load_global=T_load  initLoad_global=init_load  num=41
  Load-42 : myLibrary/Load  T_load_global=T_load  initLoad_global=init_load  num=42
  Load-43 : myLibrary/Load  T_load_global=T_load  initLoad_global=init_load  num=43
  Load-44 : myLibrary/Load  T_load_global=T_load  initLoad_global=init_load  num=44
  Load-45 : myLibrary/Load  T_load_global=T_load  initLoad_global=init_load  num=45
  Load-46 : myLibrary/Load  T_load_global=T_load  initLoad_global=init_load  num=46
  Load-47 : myLibrary/Load  T_load_global=T_load  initLoad_global=init_load  num=47
  Load-48 : myLibrary/Load  T_load_global=T_load  initLoad_global=init_load  num=48
  Load-49 : myLibrary/Load  T_load_global=T_load  initLoad_global=init_load  num=49
  Load-5 : myLibrary/Load  T_load_global=T_load  initLoad_global=init_load  num=5
  Load-50 : myLibrary/Load  T_load_global=T_load  initLoad_global=init_load  num=50
  Load-51 : myLibrary/Load  T_load_global=T_load  initLoad_global=init_load  num=51
  Load-52 : myLibrary/Load  T_load_global=T_load  initLoad_global=init_load  num=52
  Load-53 : myLibrary/Load  T_load_global=T_load  initLoad_global=init_load  num=53
  Load-54 : myLibrary/Load  T_load_global=T_load  initLoad_global=init_load  num=54
  Load-55 : myLibrary/Load  T_load_global=T_load  initLoad_global=init_load  num=55
  Load-56 : myLibrary/Load  T_load_global=T_load  initLoad_global=init_load  num=56
  Load-57 : myLibrary/Load  T_load_global=T_load  initLoad_global=init_load  num=57
  Load-58 : myLibrary/Load  T_load_global=T_load  initLoad_global=init_load  num=58
  Load-59 : myLibrary/Load  T_load_global=T_load  initLoad_global=init_load  num=59
  Load-6 : myLibrary/Load  T_load_global=T_load  initLoad_global=init_load  num=6
  Load-60 : myLibrary/Load  T_load_global=T_load  initLoad_global=init_load  num=60
  Load-61 : myLibrary/Load  T_load_global=T_load  initLoad_global=init_load  num=61
  Load-62 : myLibrary/Load  T_load_global=T_load  initLoad_global=init_load  num=62
  Load-63 : myLibrary/Load  T_load_global=T_load  initLoad_global=init_load  num=63
  Load-64 : myLibrary/Load  T_load_global=T_load  initLoad_global=init_load  num=64
  Load-65 : myLibrary/Load  T_load_global=T_load  initLoad_global=init_load  num=65
  Load-66 : myLibrary/Load  T_load_global=T_load  initLoad_global=init_load  num=66
  Load-67 : myLibrary/Load  T_load_global=T_load  initLoad_global=init_load  num=67
  Load-68 : myLibrary/Load  T_load_global=T_load  initLoad_global=init_load  num=68
  Load-69 : myLibrary/Load  T_load_global=T_load  initLoad_global=init_load  num=69
  Load-7 : myLibrary/Load  T_load_global=T_load  initLoad_global=init_load  num=7
  Load-70 : myLibrary/Load  T_load_global=T_load  initLoad_global=init_load  num=70
  Load-71 : myLibrary/Load  T_load_global=T_load  initLoad_global=init_load  num=71
  Load-72 : myLibrary/Load  T_load_global=T_load  initLoad_global=init_load  num=72
  Load-73 : myLibrary/Load  T_load_global=T_load  initLoad_global=init_load  num=73
  Load-74 : myLibrary/Load  T_load_global=T_load  initLoad_global=init_load  num=74
  Load-75 : myLibrary/Load  T_load_global=T_load  initLoad_global=init_load  num=75
  Load-76 : myLibrary/Load  T_load_global=T_load  initLoad_global=init_load  num=76
  Load-77 : myLibrary/Load  T_load_global=T_load  initLoad_global=init_load  num=77
  Load-78 : myLibrary/Load  T_load_global=T_load  initLoad_global=init_load  num=78
  Load-79 : myLibrary/Load  T_load_global=T_load  initLoad_global=init_load  num=79
  Load-8 : myLibrary/Load  T_load_global=T_load  initLoad_global=init_load  num=8
  Load-80 : myLibrary/Load  T_load_global=T_load  initLoad_global=init_load  num=80
  Load-81 : myLibrary/Load  T_load_global=T_load  initLoad_global=init_load  num=81
  Load-82 : myLibrary/Load  T_load_global=T_load  initLoad_global=init_load  num=82
  Load-83 : myLibrary/Load  T_load_global=T_load  initLoad_global=init_load  num=83
  Load-84 : myLibrary/Load  T_load_global=T_load  initLoad_global=init_load  num=84
  Load-85 : myLibrary/Load  T_load_global=T_load  initLoad_global=init_load  num=85
  Load-86 : myLibrary/Load  T_load_global=T_load  initLoad_global=init_load  num=86
  Load-87 : myLibrary/Load  T_load_global=T_load  initLoad_global=init_load  num=87
  Load-88 : myLibrary/Load  T_load_global=T_load  initLoad_global=init_load  num=88
  Load-89 : myLibrary/Load  T_load_global=T_load  initLoad_global=init_load  num=89
  Load-9 : myLibrary/Load  T_load_global=T_load  initLoad_global=init_load  num=9
  Load-90 : myLibrary/Load  T_load_global=T_load  initLoad_global=init_load  num=90
  Load-91 : myLibrary/Load  T_load_global=T_load  initLoad_global=init_load  num=91
  Mux{,1..112} (113 alike) : Mux  Inputs=2
  Power{,1..136} (137 alike) : spsPower3phInstantaneousLib/Power (3ph, Instantaneous)
  SG-1 : myLibrary/SG  num=1  init_SG_global=init_SG  initMachineBlocks=initMachineBlocks  T_SG_global=T_SG
  SG-10 : myLibrary/SG  num=10  init_SG_global=init_SG  initMachineBlocks=initMachineBlocks  T_SG_global=T_SG
  SG-11 : myLibrary/SG  num=11  init_SG_global=init_SG  initMachineBlocks=initMachineBlocks  T_SG_global=T_SG
  SG-12 : myLibrary/SG  num=12  init_SG_global=init_SG  initMachineBlocks=initMachineBlocks  T_SG_global=T_SG
  SG-13 : myLibrary/SG  num=13  init_SG_global=init_SG  initMachineBlocks=initMachineBlocks  T_SG_global=T_SG
  SG-14 : myLibrary/SG  num=14  init_SG_global=init_SG  initMachineBlocks=initMachineBlocks  T_SG_global=T_SG
  SG-15 : myLibrary/SG  num=15  init_SG_global=init_SG  initMachineBlocks=initMachineBlocks  T_SG_global=T_SG
  SG-16 : myLibrary/SG  num=16  init_SG_global=init_SG  initMachineBlocks=initMachineBlocks  T_SG_global=T_SG
  SG-17 : myLibrary/SG  num=17  init_SG_global=init_SG  initMachineBlocks=initMachineBlocks  T_SG_global=T_SG
  SG-18 : myLibrary/SG  num=18  init_SG_global=init_SG  initMachineBlocks=initMachineBlocks  T_SG_global=T_SG
  SG-19 : myLibrary/SG  num=19  init_SG_global=init_SG  initMachineBlocks=initMachineBlocks  T_SG_global=T_SG
  SG-2 : myLibrary/SG  num=2  init_SG_global=init_SG  initMachineBlocks=initMachineBlocks  T_SG_global=T_SG
  SG-20 : myLibrary/SG  num=20  init_SG_global=init_SG  initMachineBlocks=initMachineBlocks  T_SG_global=T_SG
  SG-21 : myLibrary/SG  num=21  init_SG_global=init_SG  initMachineBlocks=initMachineBlocks  T_SG_global=T_SG
  SG-22 : myLibrary/SG  num=22  init_SG_global=init_SG  initMachineBlocks=initMachineBlocks  T_SG_global=T_SG
  SG-23 : myLibrary/SG  num=23  init_SG_global=init_SG  initMachineBlocks=initMachineBlocks  T_SG_global=T_SG
  SG-24 : myLibrary/SG  num=24  init_SG_global=init_SG  initMachineBlocks=initMachineBlocks  T_SG_global=T_SG
  SG-25 : myLibrary/SG  num=25  init_SG_global=init_SG  initMachineBlocks=initMachineBlocks  T_SG_global=T_SG
  SG-26 : myLibrary/SG  num=26  init_SG_global=init_SG  initMachineBlocks=initMachineBlocks  T_SG_global=T_SG
  SG-3 : myLibrary/SG  num=3  init_SG_global=init_SG  initMachineBlocks=initMachineBlocks  T_SG_global=T_SG
  SG-4 : myLibrary/SG  num=4  init_SG_global=init_SG  initMachineBlocks=initMachineBlocks  T_SG_global=T_SG
  SG-5 : myLibrary/SG  num=5  init_SG_global=init_SG  initMachineBlocks=initMachineBlocks  T_SG_global=T_SG
  SG-6 : myLibrary/SG  num=6  init_SG_global=init_SG  initMachineBlocks=initMachineBlocks  T_SG_global=T_SG
  SG-7 : myLibrary/SG  num=7  init_SG_global=init_SG  initMachineBlocks=initMachineBlocks  T_SG_global=T_SG
  SG-8 : myLibrary/SG  num=8  init_SG_global=init_SG  initMachineBlocks=initMachineBlocks  T_SG_global=T_SG
  SG-9 : myLibrary/SG  num=9  init_SG_global=init_SG  initMachineBlocks=initMachineBlocks  T_SG_global=T_SG
  Scope{,1..225} (226 alike) : Scope
  Scope{226..227,229..230,232..233,235..236,238..239,241..242,244..245,247..248,250..251,253..254,256..257,259..260,262..263,265..266,268..269,271..272,274..275,277..278,280..281,283..284,286..287,289..290,292..293,295..296,298..299,301..302,304..305,307..308,310..311,313..314,316..317,319..320,322..323,325..326,328..329,331..332,334..335,337..338,340..341,343..344,346..347,349..350,352..353,355..356,358..359,361..362,364..365,367..368,370..371,373..374,376..377,379..380,382..383,385..386,388..389,391..392,394..395,397..398,400..401,403..404,406..407,409..410,412..413,415..416,418..419,421..422,424..425,427..428,430..431,433..434,436..437,439..440,442..443,445..446,448..449,451..452,454..455,457..458,460..461,463..464,466..467,469..470,472..473,475..476,478..479,481..482,484..485,487..488,490..491,493..494,496..497,499..500,502..503,505..506,508..509,511..512,514..515,517..518,520..521,523..524,526..527,529..530,532..533,535..536,538..539,541..542,544..545,547..548,550..551,553..554,556..557,559..560,562..563,565..566,568..569,571..572,574..575,577..578,580..581,583..584,586..587,589..590,592..593,595..596,598..599,601..602,604..605,607..608,610..611,613..614,616..617,619..620,622..623,625..626,628..629,631..632,634..635} (274 alike) : Display
  Scope{228,231,234,237,240,243,246,249,252,255,258,261,264,267,270,273,276,279,282,285,288,291,294,297,300,303,306,309,312,315,318,321,324,327,330,333,336,339,342,345,348,351,354,357,360,363,366,369,372,375,378,381,384,387,390,393,396,399,402,405,408,411,414,417,420,423,426,429,432,435,438,441,444,447,450,453,456,459,462,465,468,471,474,477,480,483,486,489,492,495,498,501,504,507,510,513,516,519,522,525,528,531,534,537,540,543,546,549,552,555,558,561,564,567,570,573,576,579,582,585,588,591,594,597,600,603,606,609,612,615,618,621,624,627,630,633,636} (137 alike) : Scope  NumInputPorts=2
  To WorkspaceGFOL_RL10_w : ToWorkspace  VariableName=GFOL_RL10_w  SampleTime=sim_config.Tsample
  To WorkspaceGFOL_RL1_w : ToWorkspace  VariableName=GFOL_RL1_w  SampleTime=sim_config.Tsample
  To WorkspaceGFOL_RL2_w : ToWorkspace  VariableName=GFOL_RL2_w  SampleTime=sim_config.Tsample
  To WorkspaceGFOL_RL3_w : ToWorkspace  VariableName=GFOL_RL3_w  SampleTime=sim_config.Tsample
  To WorkspaceGFOL_RL4_w : ToWorkspace  VariableName=GFOL_RL4_w  SampleTime=sim_config.Tsample
  To WorkspaceGFOL_RL5_w : ToWorkspace  VariableName=GFOL_RL5_w  SampleTime=sim_config.Tsample
  To WorkspaceGFOL_RL6_w : ToWorkspace  VariableName=GFOL_RL6_w  SampleTime=sim_config.Tsample
  To WorkspaceGFOL_RL7_w : ToWorkspace  VariableName=GFOL_RL7_w  SampleTime=sim_config.Tsample
  To WorkspaceGFOL_RL8_w : ToWorkspace  VariableName=GFOL_RL8_w  SampleTime=sim_config.Tsample
  To WorkspaceGFOL_RL9_w : ToWorkspace  VariableName=GFOL_RL9_w  SampleTime=sim_config.Tsample
  To WorkspaceGFOR11_w : ToWorkspace  VariableName=GFOR11_w  SampleTime=sim_config.Tsample
  To WorkspaceGFOR12_w : ToWorkspace  VariableName=GFOR12_w  SampleTime=sim_config.Tsample
  To WorkspaceGFOR13_w : ToWorkspace  VariableName=GFOR13_w  SampleTime=sim_config.Tsample
  To WorkspaceGFOR14_w : ToWorkspace  VariableName=GFOR14_w  SampleTime=sim_config.Tsample
  To WorkspaceGFOR15_w : ToWorkspace  VariableName=GFOR15_w  SampleTime=sim_config.Tsample
  To WorkspaceGFOR16_w : ToWorkspace  VariableName=GFOR16_w  SampleTime=sim_config.Tsample
  To WorkspaceGFOR17_w : ToWorkspace  VariableName=GFOR17_w  SampleTime=sim_config.Tsample
  To WorkspaceGFOR18_w : ToWorkspace  VariableName=GFOR18_w  SampleTime=sim_config.Tsample
  To WorkspaceGFOR19_w : ToWorkspace  VariableName=GFOR19_w  SampleTime=sim_config.Tsample
  To WorkspaceGFOR20_w : ToWorkspace  VariableName=GFOR20_w  SampleTime=sim_config.Tsample
  To WorkspaceSG10_w : ToWorkspace  VariableName=SG10_w  SampleTime=sim_config.Tsample
  To WorkspaceSG11_w : ToWorkspace  VariableName=SG11_w  SampleTime=sim_config.Tsample
  To WorkspaceSG12_w : ToWorkspace  VariableName=SG12_w  SampleTime=sim_config.Tsample
  To WorkspaceSG13_w : ToWorkspace  VariableName=SG13_w  SampleTime=sim_config.Tsample
  To WorkspaceSG14_w : ToWorkspace  VariableName=SG14_w  SampleTime=sim_config.Tsample
  To WorkspaceSG15_w : ToWorkspace  VariableName=SG15_w  SampleTime=sim_config.Tsample
  To WorkspaceSG16_w : ToWorkspace  VariableName=SG16_w  SampleTime=sim_config.Tsample
  To WorkspaceSG17_w : ToWorkspace  VariableName=SG17_w  SampleTime=sim_config.Tsample
  To WorkspaceSG18_w : ToWorkspace  VariableName=SG18_w  SampleTime=sim_config.Tsample
  To WorkspaceSG19_w : ToWorkspace  VariableName=SG19_w  SampleTime=sim_config.Tsample
  To WorkspaceSG1_w : ToWorkspace  VariableName=SG1_w  SampleTime=sim_config.Tsample
  To WorkspaceSG20_w : ToWorkspace  VariableName=SG20_w  SampleTime=sim_config.Tsample
  To WorkspaceSG21_w : ToWorkspace  VariableName=SG21_w  SampleTime=sim_config.Tsample
  To WorkspaceSG22_w : ToWorkspace  VariableName=SG22_w  SampleTime=sim_config.Tsample
  To WorkspaceSG23_w : ToWorkspace  VariableName=SG23_w  SampleTime=sim_config.Tsample
  To WorkspaceSG24_w : ToWorkspace  VariableName=SG24_w  SampleTime=sim_config.Tsample
  To WorkspaceSG25_w : ToWorkspace  VariableName=SG25_w  SampleTime=sim_config.Tsample
  To WorkspaceSG26_w : ToWorkspace  VariableName=SG26_w  SampleTime=sim_config.Tsample
  To WorkspaceSG2_w : ToWorkspace  VariableName=SG2_w  SampleTime=sim_config.Tsample
  To WorkspaceSG3_w : ToWorkspace  VariableName=SG3_w  SampleTime=sim_config.Tsample
  To WorkspaceSG4_w : ToWorkspace  VariableName=SG4_w  SampleTime=sim_config.Tsample
  To WorkspaceSG5_w : ToWorkspace  VariableName=SG5_w  SampleTime=sim_config.Tsample
  To WorkspaceSG6_w : ToWorkspace  VariableName=SG6_w  SampleTime=sim_config.Tsample
  To WorkspaceSG7_w : ToWorkspace  VariableName=SG7_w  SampleTime=sim_config.Tsample
  To WorkspaceSG8_w : ToWorkspace  VariableName=SG8_w  SampleTime=sim_config.Tsample
  To WorkspaceSG9_w : ToWorkspace  VariableName=SG9_w  SampleTime=sim_config.Tsample
  To Workspace_I_Load10_d : ToWorkspace  VariableName=I_Load10_d  SampleTime=sim_config.Tsample
  To Workspace_I_Load10_q : ToWorkspace  VariableName=I_Load10_q  SampleTime=sim_config.Tsample
  To Workspace_I_Load11_d : ToWorkspace  VariableName=I_Load11_d  SampleTime=sim_config.Tsample
  To Workspace_I_Load11_q : ToWorkspace  VariableName=I_Load11_q  SampleTime=sim_config.Tsample
  To Workspace_I_Load12_d : ToWorkspace  VariableName=I_Load12_d  SampleTime=sim_config.Tsample
  To Workspace_I_Load12_q : ToWorkspace  VariableName=I_Load12_q  SampleTime=sim_config.Tsample
  To Workspace_I_Load13_d : ToWorkspace  VariableName=I_Load13_d  SampleTime=sim_config.Tsample
  To Workspace_I_Load13_q : ToWorkspace  VariableName=I_Load13_q  SampleTime=sim_config.Tsample
  To Workspace_I_Load14_d : ToWorkspace  VariableName=I_Load14_d  SampleTime=sim_config.Tsample
  To Workspace_I_Load14_q : ToWorkspace  VariableName=I_Load14_q  SampleTime=sim_config.Tsample
  To Workspace_I_Load15_d : ToWorkspace  VariableName=I_Load15_d  SampleTime=sim_config.Tsample
  To Workspace_I_Load15_q : ToWorkspace  VariableName=I_Load15_q  SampleTime=sim_config.Tsample
  To Workspace_I_Load16_d : ToWorkspace  VariableName=I_Load16_d  SampleTime=sim_config.Tsample
  To Workspace_I_Load16_q : ToWorkspace  VariableName=I_Load16_q  SampleTime=sim_config.Tsample
  To Workspace_I_Load17_d : ToWorkspace  VariableName=I_Load17_d  SampleTime=sim_config.Tsample
  To Workspace_I_Load17_q : ToWorkspace  VariableName=I_Load17_q  SampleTime=sim_config.Tsample
  To Workspace_I_Load18_d : ToWorkspace  VariableName=I_Load18_d  SampleTime=sim_config.Tsample
  To Workspace_I_Load18_q : ToWorkspace  VariableName=I_Load18_q  SampleTime=sim_config.Tsample
  To Workspace_I_Load19_d : ToWorkspace  VariableName=I_Load19_d  SampleTime=sim_config.Tsample
  To Workspace_I_Load19_q : ToWorkspace  VariableName=I_Load19_q  SampleTime=sim_config.Tsample
  To Workspace_I_Load1_d : ToWorkspace  VariableName=I_Load1_d  SampleTime=sim_config.Tsample
  To Workspace_I_Load1_q : ToWorkspace  VariableName=I_Load1_q  SampleTime=sim_config.Tsample
  To Workspace_I_Load20_d : ToWorkspace  VariableName=I_Load20_d  SampleTime=sim_config.Tsample
  To Workspace_I_Load20_q : ToWorkspace  VariableName=I_Load20_q  SampleTime=sim_config.Tsample
  To Workspace_I_Load21_d : ToWorkspace  VariableName=I_Load21_d  SampleTime=sim_config.Tsample
  To Workspace_I_Load21_q : ToWorkspace  VariableName=I_Load21_q  SampleTime=sim_config.Tsample
  To Workspace_I_Load22_d : ToWorkspace  VariableName=I_Load22_d  SampleTime=sim_config.Tsample
  To Workspace_I_Load22_q : ToWorkspace  VariableName=I_Load22_q  SampleTime=sim_config.Tsample
  To Workspace_I_Load23_d : ToWorkspace  VariableName=I_Load23_d  SampleTime=sim_config.Tsample
  To Workspace_I_Load23_q : ToWorkspace  VariableName=I_Load23_q  SampleTime=sim_config.Tsample
  To Workspace_I_Load24_d : ToWorkspace  VariableName=I_Load24_d  SampleTime=sim_config.Tsample
  To Workspace_I_Load24_q : ToWorkspace  VariableName=I_Load24_q  SampleTime=sim_config.Tsample
  To Workspace_I_Load25_d : ToWorkspace  VariableName=I_Load25_d  SampleTime=sim_config.Tsample
  To Workspace_I_Load25_q : ToWorkspace  VariableName=I_Load25_q  SampleTime=sim_config.Tsample
  To Workspace_I_Load26_d : ToWorkspace  VariableName=I_Load26_d  SampleTime=sim_config.Tsample
  To Workspace_I_Load26_q : ToWorkspace  VariableName=I_Load26_q  SampleTime=sim_config.Tsample
  To Workspace_I_Load27_d : ToWorkspace  VariableName=I_Load27_d  SampleTime=sim_config.Tsample
  To Workspace_I_Load27_q : ToWorkspace  VariableName=I_Load27_q  SampleTime=sim_config.Tsample
  To Workspace_I_Load28_d : ToWorkspace  VariableName=I_Load28_d  SampleTime=sim_config.Tsample
  To Workspace_I_Load28_q : ToWorkspace  VariableName=I_Load28_q  SampleTime=sim_config.Tsample
  To Workspace_I_Load29_d : ToWorkspace  VariableName=I_Load29_d  SampleTime=sim_config.Tsample
  To Workspace_I_Load29_q : ToWorkspace  VariableName=I_Load29_q  SampleTime=sim_config.Tsample
  To Workspace_I_Load2_d : ToWorkspace  VariableName=I_Load2_d  SampleTime=sim_config.Tsample
  To Workspace_I_Load2_q : ToWorkspace  VariableName=I_Load2_q  SampleTime=sim_config.Tsample
  To Workspace_I_Load30_d : ToWorkspace  VariableName=I_Load30_d  SampleTime=sim_config.Tsample
  To Workspace_I_Load30_q : ToWorkspace  VariableName=I_Load30_q  SampleTime=sim_config.Tsample
  To Workspace_I_Load31_d : ToWorkspace  VariableName=I_Load31_d  SampleTime=sim_config.Tsample
  To Workspace_I_Load31_q : ToWorkspace  VariableName=I_Load31_q  SampleTime=sim_config.Tsample
  To Workspace_I_Load32_d : ToWorkspace  VariableName=I_Load32_d  SampleTime=sim_config.Tsample
  To Workspace_I_Load32_q : ToWorkspace  VariableName=I_Load32_q  SampleTime=sim_config.Tsample
  To Workspace_I_Load33_d : ToWorkspace  VariableName=I_Load33_d  SampleTime=sim_config.Tsample
  To Workspace_I_Load33_q : ToWorkspace  VariableName=I_Load33_q  SampleTime=sim_config.Tsample
  To Workspace_I_Load34_d : ToWorkspace  VariableName=I_Load34_d  SampleTime=sim_config.Tsample
  To Workspace_I_Load34_q : ToWorkspace  VariableName=I_Load34_q  SampleTime=sim_config.Tsample
  To Workspace_I_Load35_d : ToWorkspace  VariableName=I_Load35_d  SampleTime=sim_config.Tsample
  To Workspace_I_Load35_q : ToWorkspace  VariableName=I_Load35_q  SampleTime=sim_config.Tsample
  To Workspace_I_Load36_d : ToWorkspace  VariableName=I_Load36_d  SampleTime=sim_config.Tsample
  To Workspace_I_Load36_q : ToWorkspace  VariableName=I_Load36_q  SampleTime=sim_config.Tsample
  To Workspace_I_Load37_d : ToWorkspace  VariableName=I_Load37_d  SampleTime=sim_config.Tsample
  To Workspace_I_Load37_q : ToWorkspace  VariableName=I_Load37_q  SampleTime=sim_config.Tsample
  To Workspace_I_Load38_d : ToWorkspace  VariableName=I_Load38_d  SampleTime=sim_config.Tsample
  To Workspace_I_Load38_q : ToWorkspace  VariableName=I_Load38_q  SampleTime=sim_config.Tsample
  To Workspace_I_Load39_d : ToWorkspace  VariableName=I_Load39_d  SampleTime=sim_config.Tsample
  To Workspace_I_Load39_q : ToWorkspace  VariableName=I_Load39_q  SampleTime=sim_config.Tsample
  To Workspace_I_Load3_d : ToWorkspace  VariableName=I_Load3_d  SampleTime=sim_config.Tsample
  To Workspace_I_Load3_q : ToWorkspace  VariableName=I_Load3_q  SampleTime=sim_config.Tsample
  To Workspace_I_Load40_d : ToWorkspace  VariableName=I_Load40_d  SampleTime=sim_config.Tsample
  To Workspace_I_Load40_q : ToWorkspace  VariableName=I_Load40_q  SampleTime=sim_config.Tsample
  To Workspace_I_Load41_d : ToWorkspace  VariableName=I_Load41_d  SampleTime=sim_config.Tsample
  To Workspace_I_Load41_q : ToWorkspace  VariableName=I_Load41_q  SampleTime=sim_config.Tsample
  To Workspace_I_Load42_d : ToWorkspace  VariableName=I_Load42_d  SampleTime=sim_config.Tsample
  To Workspace_I_Load42_q : ToWorkspace  VariableName=I_Load42_q  SampleTime=sim_config.Tsample
  To Workspace_I_Load43_d : ToWorkspace  VariableName=I_Load43_d  SampleTime=sim_config.Tsample
  To Workspace_I_Load43_q : ToWorkspace  VariableName=I_Load43_q  SampleTime=sim_config.Tsample
  To Workspace_I_Load44_d : ToWorkspace  VariableName=I_Load44_d  SampleTime=sim_config.Tsample
  To Workspace_I_Load44_q : ToWorkspace  VariableName=I_Load44_q  SampleTime=sim_config.Tsample
  To Workspace_I_Load45_d : ToWorkspace  VariableName=I_Load45_d  SampleTime=sim_config.Tsample
  To Workspace_I_Load45_q : ToWorkspace  VariableName=I_Load45_q  SampleTime=sim_config.Tsample
  To Workspace_I_Load46_d : ToWorkspace  VariableName=I_Load46_d  SampleTime=sim_config.Tsample
  To Workspace_I_Load46_q : ToWorkspace  VariableName=I_Load46_q  SampleTime=sim_config.Tsample
  To Workspace_I_Load47_d : ToWorkspace  VariableName=I_Load47_d  SampleTime=sim_config.Tsample
  To Workspace_I_Load47_q : ToWorkspace  VariableName=I_Load47_q  SampleTime=sim_config.Tsample
  To Workspace_I_Load48_d : ToWorkspace  VariableName=I_Load48_d  SampleTime=sim_config.Tsample
  To Workspace_I_Load48_q : ToWorkspace  VariableName=I_Load48_q  SampleTime=sim_config.Tsample
  To Workspace_I_Load49_d : ToWorkspace  VariableName=I_Load49_d  SampleTime=sim_config.Tsample
  To Workspace_I_Load49_q : ToWorkspace  VariableName=I_Load49_q  SampleTime=sim_config.Tsample
  To Workspace_I_Load4_d : ToWorkspace  VariableName=I_Load4_d  SampleTime=sim_config.Tsample
  To Workspace_I_Load4_q : ToWorkspace  VariableName=I_Load4_q  SampleTime=sim_config.Tsample
  To Workspace_I_Load50_d : ToWorkspace  VariableName=I_Load50_d  SampleTime=sim_config.Tsample
  To Workspace_I_Load50_q : ToWorkspace  VariableName=I_Load50_q  SampleTime=sim_config.Tsample
  To Workspace_I_Load51_d : ToWorkspace  VariableName=I_Load51_d  SampleTime=sim_config.Tsample
  To Workspace_I_Load51_q : ToWorkspace  VariableName=I_Load51_q  SampleTime=sim_config.Tsample
  To Workspace_I_Load52_d : ToWorkspace  VariableName=I_Load52_d  SampleTime=sim_config.Tsample
  To Workspace_I_Load52_q : ToWorkspace  VariableName=I_Load52_q  SampleTime=sim_config.Tsample
  To Workspace_I_Load53_d : ToWorkspace  VariableName=I_Load53_d  SampleTime=sim_config.Tsample
  To Workspace_I_Load53_q : ToWorkspace  VariableName=I_Load53_q  SampleTime=sim_config.Tsample
  To Workspace_I_Load54_d : ToWorkspace  VariableName=I_Load54_d  SampleTime=sim_config.Tsample
  To Workspace_I_Load54_q : ToWorkspace  VariableName=I_Load54_q  SampleTime=sim_config.Tsample
  To Workspace_I_Load55_d : ToWorkspace  VariableName=I_Load55_d  SampleTime=sim_config.Tsample
  To Workspace_I_Load55_q : ToWorkspace  VariableName=I_Load55_q  SampleTime=sim_config.Tsample
  To Workspace_I_Load56_d : ToWorkspace  VariableName=I_Load56_d  SampleTime=sim_config.Tsample
  To Workspace_I_Load56_q : ToWorkspace  VariableName=I_Load56_q  SampleTime=sim_config.Tsample
  To Workspace_I_Load57_d : ToWorkspace  VariableName=I_Load57_d  SampleTime=sim_config.Tsample
  To Workspace_I_Load57_q : ToWorkspace  VariableName=I_Load57_q  SampleTime=sim_config.Tsample
  To Workspace_I_Load58_d : ToWorkspace  VariableName=I_Load58_d  SampleTime=sim_config.Tsample
  To Workspace_I_Load58_q : ToWorkspace  VariableName=I_Load58_q  SampleTime=sim_config.Tsample
  To Workspace_I_Load59_d : ToWorkspace  VariableName=I_Load59_d  SampleTime=sim_config.Tsample
  To Workspace_I_Load59_q : ToWorkspace  VariableName=I_Load59_q  SampleTime=sim_config.Tsample
  To Workspace_I_Load5_d : ToWorkspace  VariableName=I_Load5_d  SampleTime=sim_config.Tsample
  To Workspace_I_Load5_q : ToWorkspace  VariableName=I_Load5_q  SampleTime=sim_config.Tsample
  To Workspace_I_Load60_d : ToWorkspace  VariableName=I_Load60_d  SampleTime=sim_config.Tsample
  To Workspace_I_Load60_q : ToWorkspace  VariableName=I_Load60_q  SampleTime=sim_config.Tsample
  To Workspace_I_Load61_d : ToWorkspace  VariableName=I_Load61_d  SampleTime=sim_config.Tsample
  To Workspace_I_Load61_q : ToWorkspace  VariableName=I_Load61_q  SampleTime=sim_config.Tsample
  To Workspace_I_Load62_d : ToWorkspace  VariableName=I_Load62_d  SampleTime=sim_config.Tsample
  To Workspace_I_Load62_q : ToWorkspace  VariableName=I_Load62_q  SampleTime=sim_config.Tsample
  To Workspace_I_Load63_d : ToWorkspace  VariableName=I_Load63_d  SampleTime=sim_config.Tsample
  To Workspace_I_Load63_q : ToWorkspace  VariableName=I_Load63_q  SampleTime=sim_config.Tsample
  To Workspace_I_Load64_d : ToWorkspace  VariableName=I_Load64_d  SampleTime=sim_config.Tsample
  To Workspace_I_Load64_q : ToWorkspace  VariableName=I_Load64_q  SampleTime=sim_config.Tsample
  To Workspace_I_Load65_d : ToWorkspace  VariableName=I_Load65_d  SampleTime=sim_config.Tsample
  To Workspace_I_Load65_q : ToWorkspace  VariableName=I_Load65_q  SampleTime=sim_config.Tsample
  To Workspace_I_Load66_d : ToWorkspace  VariableName=I_Load66_d  SampleTime=sim_config.Tsample
  To Workspace_I_Load66_q : ToWorkspace  VariableName=I_Load66_q  SampleTime=sim_config.Tsample
  To Workspace_I_Load67_d : ToWorkspace  VariableName=I_Load67_d  SampleTime=sim_config.Tsample
  To Workspace_I_Load67_q : ToWorkspace  VariableName=I_Load67_q  SampleTime=sim_config.Tsample
  To Workspace_I_Load68_d : ToWorkspace  VariableName=I_Load68_d  SampleTime=sim_config.Tsample
  To Workspace_I_Load68_q : ToWorkspace  VariableName=I_Load68_q  SampleTime=sim_config.Tsample
  To Workspace_I_Load69_d : ToWorkspace  VariableName=I_Load69_d  SampleTime=sim_config.Tsample
  To Workspace_I_Load69_q : ToWorkspace  VariableName=I_Load69_q  SampleTime=sim_config.Tsample
  To Workspace_I_Load6_d : ToWorkspace  VariableName=I_Load6_d  SampleTime=sim_config.Tsample
  To Workspace_I_Load6_q : ToWorkspace  VariableName=I_Load6_q  SampleTime=sim_config.Tsample
  To Workspace_I_Load70_d : ToWorkspace  VariableName=I_Load70_d  SampleTime=sim_config.Tsample
  To Workspace_I_Load70_q : ToWorkspace  VariableName=I_Load70_q  SampleTime=sim_config.Tsample
  To Workspace_I_Load71_d : ToWorkspace  VariableName=I_Load71_d  SampleTime=sim_config.Tsample
  To Workspace_I_Load71_q : ToWorkspace  VariableName=I_Load71_q  SampleTime=sim_config.Tsample
  To Workspace_I_Load72_d : ToWorkspace  VariableName=I_Load72_d  SampleTime=sim_config.Tsample
  To Workspace_I_Load72_q : ToWorkspace  VariableName=I_Load72_q  SampleTime=sim_config.Tsample
  To Workspace_I_Load73_d : ToWorkspace  VariableName=I_Load73_d  SampleTime=sim_config.Tsample
  To Workspace_I_Load73_q : ToWorkspace  VariableName=I_Load73_q  SampleTime=sim_config.Tsample
  To Workspace_I_Load74_d : ToWorkspace  VariableName=I_Load74_d  SampleTime=sim_config.Tsample
  To Workspace_I_Load74_q : ToWorkspace  VariableName=I_Load74_q  SampleTime=sim_config.Tsample
  To Workspace_I_Load75_d : ToWorkspace  VariableName=I_Load75_d  SampleTime=sim_config.Tsample
  To Workspace_I_Load75_q : ToWorkspace  VariableName=I_Load75_q  SampleTime=sim_config.Tsample
  To Workspace_I_Load76_d : ToWorkspace  VariableName=I_Load76_d  SampleTime=sim_config.Tsample
  To Workspace_I_Load76_q : ToWorkspace  VariableName=I_Load76_q  SampleTime=sim_config.Tsample
  To Workspace_I_Load77_d : ToWorkspace  VariableName=I_Load77_d  SampleTime=sim_config.Tsample
  To Workspace_I_Load77_q : ToWorkspace  VariableName=I_Load77_q  SampleTime=sim_config.Tsample
  To Workspace_I_Load78_d : ToWorkspace  VariableName=I_Load78_d  SampleTime=sim_config.Tsample
  To Workspace_I_Load78_q : ToWorkspace  VariableName=I_Load78_q  SampleTime=sim_config.Tsample
  To Workspace_I_Load79_d : ToWorkspace  VariableName=I_Load79_d  SampleTime=sim_config.Tsample
  To Workspace_I_Load79_q : ToWorkspace  VariableName=I_Load79_q  SampleTime=sim_config.Tsample
  To Workspace_I_Load7_d : ToWorkspace  VariableName=I_Load7_d  SampleTime=sim_config.Tsample
  To Workspace_I_Load7_q : ToWorkspace  VariableName=I_Load7_q  SampleTime=sim_config.Tsample
  To Workspace_I_Load80_d : ToWorkspace  VariableName=I_Load80_d  SampleTime=sim_config.Tsample
  To Workspace_I_Load80_q : ToWorkspace  VariableName=I_Load80_q  SampleTime=sim_config.Tsample
  To Workspace_I_Load81_d : ToWorkspace  VariableName=I_Load81_d  SampleTime=sim_config.Tsample
  To Workspace_I_Load81_q : ToWorkspace  VariableName=I_Load81_q  SampleTime=sim_config.Tsample
  To Workspace_I_Load82_d : ToWorkspace  VariableName=I_Load82_d  SampleTime=sim_config.Tsample
  To Workspace_I_Load82_q : ToWorkspace  VariableName=I_Load82_q  SampleTime=sim_config.Tsample
  To Workspace_I_Load83_d : ToWorkspace  VariableName=I_Load83_d  SampleTime=sim_config.Tsample
  To Workspace_I_Load83_q : ToWorkspace  VariableName=I_Load83_q  SampleTime=sim_config.Tsample
  To Workspace_I_Load84_d : ToWorkspace  VariableName=I_Load84_d  SampleTime=sim_config.Tsample
  To Workspace_I_Load84_q : ToWorkspace  VariableName=I_Load84_q  SampleTime=sim_config.Tsample
  To Workspace_I_Load85_d : ToWorkspace  VariableName=I_Load85_d  SampleTime=sim_config.Tsample
  To Workspace_I_Load85_q : ToWorkspace  VariableName=I_Load85_q  SampleTime=sim_config.Tsample
  To Workspace_I_Load86_d : ToWorkspace  VariableName=I_Load86_d  SampleTime=sim_config.Tsample
  To Workspace_I_Load86_q : ToWorkspace  VariableName=I_Load86_q  SampleTime=sim_config.Tsample
  To Workspace_I_Load87_d : ToWorkspace  VariableName=I_Load87_d  SampleTime=sim_config.Tsample
  To Workspace_I_Load87_q : ToWorkspace  VariableName=I_Load87_q  SampleTime=sim_config.Tsample
  To Workspace_I_Load88_d : ToWorkspace  VariableName=I_Load88_d  SampleTime=sim_config.Tsample
  To Workspace_I_Load88_q : ToWorkspace  VariableName=I_Load88_q  SampleTime=sim_config.Tsample
  To Workspace_I_Load89_d : ToWorkspace  VariableName=I_Load89_d  SampleTime=sim_config.Tsample
  To Workspace_I_Load89_q : ToWorkspace  VariableName=I_Load89_q  SampleTime=sim_config.Tsample
  To Workspace_I_Load8_d : ToWorkspace  VariableName=I_Load8_d  SampleTime=sim_config.Tsample
  To Workspace_I_Load8_q : ToWorkspace  VariableName=I_Load8_q  SampleTime=sim_config.Tsample
  To Workspace_I_Load90_d : ToWorkspace  VariableName=I_Load90_d  SampleTime=sim_config.Tsample
  To Workspace_I_Load90_q : ToWorkspace  VariableName=I_Load90_q  SampleTime=sim_config.Tsample
  To Workspace_I_Load91_d : ToWorkspace  VariableName=I_Load91_d  SampleTime=sim_config.Tsample
  To Workspace_I_Load91_q : ToWorkspace  VariableName=I_Load91_q  SampleTime=sim_config.Tsample
  To Workspace_I_Load9_d : ToWorkspace  VariableName=I_Load9_d  SampleTime=sim_config.Tsample
  To Workspace_I_Load9_q : ToWorkspace  VariableName=I_Load9_q  SampleTime=sim_config.Tsample
  To Workspace_I_SG10_d : ToWorkspace  VariableName=I_SG10_d  SampleTime=sim_config.Tsample
  To Workspace_I_SG10_q : ToWorkspace  VariableName=I_SG10_q  SampleTime=sim_config.Tsample
  To Workspace_I_SG11_d : ToWorkspace  VariableName=I_SG11_d  SampleTime=sim_config.Tsample
  To Workspace_I_SG11_q : ToWorkspace  VariableName=I_SG11_q  SampleTime=sim_config.Tsample
  To Workspace_I_SG12_d : ToWorkspace  VariableName=I_SG12_d  SampleTime=sim_config.Tsample
  To Workspace_I_SG12_q : ToWorkspace  VariableName=I_SG12_q  SampleTime=sim_config.Tsample
  To Workspace_I_SG13_d : ToWorkspace  VariableName=I_SG13_d  SampleTime=sim_config.Tsample
  To Workspace_I_SG13_q : ToWorkspace  VariableName=I_SG13_q  SampleTime=sim_config.Tsample
  To Workspace_I_SG14_d : ToWorkspace  VariableName=I_SG14_d  SampleTime=sim_config.Tsample
  To Workspace_I_SG14_q : ToWorkspace  VariableName=I_SG14_q  SampleTime=sim_config.Tsample
  To Workspace_I_SG15_d : ToWorkspace  VariableName=I_SG15_d  SampleTime=sim_config.Tsample
  To Workspace_I_SG15_q : ToWorkspace  VariableName=I_SG15_q  SampleTime=sim_config.Tsample
  To Workspace_I_SG16_d : ToWorkspace  VariableName=I_SG16_d  SampleTime=sim_config.Tsample
  To Workspace_I_SG16_q : ToWorkspace  VariableName=I_SG16_q  SampleTime=sim_config.Tsample
  To Workspace_I_SG17_d : ToWorkspace  VariableName=I_SG17_d  SampleTime=sim_config.Tsample
  To Workspace_I_SG17_q : ToWorkspace  VariableName=I_SG17_q  SampleTime=sim_config.Tsample
  To Workspace_I_SG18_d : ToWorkspace  VariableName=I_SG18_d  SampleTime=sim_config.Tsample
  To Workspace_I_SG18_q : ToWorkspace  VariableName=I_SG18_q  SampleTime=sim_config.Tsample
  To Workspace_I_SG19_d : ToWorkspace  VariableName=I_SG19_d  SampleTime=sim_config.Tsample
  To Workspace_I_SG19_q : ToWorkspace  VariableName=I_SG19_q  SampleTime=sim_config.Tsample
  To Workspace_I_SG1_d : ToWorkspace  VariableName=I_SG1_d  SampleTime=sim_config.Tsample
  To Workspace_I_SG1_q : ToWorkspace  VariableName=I_SG1_q  SampleTime=sim_config.Tsample
  To Workspace_I_SG20_d : ToWorkspace  VariableName=I_SG20_d  SampleTime=sim_config.Tsample
  To Workspace_I_SG20_q : ToWorkspace  VariableName=I_SG20_q  SampleTime=sim_config.Tsample
  To Workspace_I_SG21_d : ToWorkspace  VariableName=I_SG21_d  SampleTime=sim_config.Tsample
  To Workspace_I_SG21_q : ToWorkspace  VariableName=I_SG21_q  SampleTime=sim_config.Tsample
  To Workspace_I_SG22_d : ToWorkspace  VariableName=I_SG22_d  SampleTime=sim_config.Tsample
  To Workspace_I_SG22_q : ToWorkspace  VariableName=I_SG22_q  SampleTime=sim_config.Tsample
  To Workspace_I_SG23_d : ToWorkspace  VariableName=I_SG23_d  SampleTime=sim_config.Tsample
  To Workspace_I_SG23_q : ToWorkspace  VariableName=I_SG23_q  SampleTime=sim_config.Tsample
  To Workspace_I_SG24_d : ToWorkspace  VariableName=I_SG24_d  SampleTime=sim_config.Tsample
  To Workspace_I_SG24_q : ToWorkspace  VariableName=I_SG24_q  SampleTime=sim_config.Tsample
  To Workspace_I_SG25_d : ToWorkspace  VariableName=I_SG25_d  SampleTime=sim_config.Tsample
  To Workspace_I_SG25_q : ToWorkspace  VariableName=I_SG25_q  SampleTime=sim_config.Tsample
  To Workspace_I_SG26_d : ToWorkspace  VariableName=I_SG26_d  SampleTime=sim_config.Tsample
  To Workspace_I_SG26_q : ToWorkspace  VariableName=I_SG26_q  SampleTime=sim_config.Tsample
  To Workspace_I_SG2_d : ToWorkspace  VariableName=I_SG2_d  SampleTime=sim_config.Tsample
  To Workspace_I_SG2_q : ToWorkspace  VariableName=I_SG2_q  SampleTime=sim_config.Tsample
  To Workspace_I_SG3_d : ToWorkspace  VariableName=I_SG3_d  SampleTime=sim_config.Tsample
  To Workspace_I_SG3_q : ToWorkspace  VariableName=I_SG3_q  SampleTime=sim_config.Tsample
  To Workspace_I_SG4_d : ToWorkspace  VariableName=I_SG4_d  SampleTime=sim_config.Tsample
  To Workspace_I_SG4_q : ToWorkspace  VariableName=I_SG4_q  SampleTime=sim_config.Tsample
  To Workspace_I_SG5_d : ToWorkspace  VariableName=I_SG5_d  SampleTime=sim_config.Tsample
  To Workspace_I_SG5_q : ToWorkspace  VariableName=I_SG5_q  SampleTime=sim_config.Tsample
  To Workspace_I_SG6_d : ToWorkspace  VariableName=I_SG6_d  SampleTime=sim_config.Tsample
  To Workspace_I_SG6_q : ToWorkspace  VariableName=I_SG6_q  SampleTime=sim_config.Tsample
  To Workspace_I_SG7_d : ToWorkspace  VariableName=I_SG7_d  SampleTime=sim_config.Tsample
  To Workspace_I_SG7_q : ToWorkspace  VariableName=I_SG7_q  SampleTime=sim_config.Tsample
  To Workspace_I_SG8_d : ToWorkspace  VariableName=I_SG8_d  SampleTime=sim_config.Tsample
  To Workspace_I_SG8_q : ToWorkspace  VariableName=I_SG8_q  SampleTime=sim_config.Tsample
  To Workspace_I_SG9_d : ToWorkspace  VariableName=I_SG9_d  SampleTime=sim_config.Tsample
  To Workspace_I_SG9_q : ToWorkspace  VariableName=I_SG9_q  SampleTime=sim_config.Tsample
  To Workspace_I_VSC10_d : ToWorkspace  VariableName=I_VSC10_d  SampleTime=sim_config.Tsample
  To Workspace_I_VSC10_q : ToWorkspace  VariableName=I_VSC10_q  SampleTime=sim_config.Tsample
  To Workspace_I_VSC11_d : ToWorkspace  VariableName=I_VSC11_d  SampleTime=sim_config.Tsample
  To Workspace_I_VSC11_q : ToWorkspace  VariableName=I_VSC11_q  SampleTime=sim_config.Tsample
  To Workspace_I_VSC12_d : ToWorkspace  VariableName=I_VSC12_d  SampleTime=sim_config.Tsample
  To Workspace_I_VSC12_q : ToWorkspace  VariableName=I_VSC12_q  SampleTime=sim_config.Tsample
  To Workspace_I_VSC13_d : ToWorkspace  VariableName=I_VSC13_d  SampleTime=sim_config.Tsample
  To Workspace_I_VSC13_q : ToWorkspace  VariableName=I_VSC13_q  SampleTime=sim_config.Tsample
  To Workspace_I_VSC14_d : ToWorkspace  VariableName=I_VSC14_d  SampleTime=sim_config.Tsample
  To Workspace_I_VSC14_q : ToWorkspace  VariableName=I_VSC14_q  SampleTime=sim_config.Tsample
  To Workspace_I_VSC15_d : ToWorkspace  VariableName=I_VSC15_d  SampleTime=sim_config.Tsample
  To Workspace_I_VSC15_q : ToWorkspace  VariableName=I_VSC15_q  SampleTime=sim_config.Tsample
  To Workspace_I_VSC16_d : ToWorkspace  VariableName=I_VSC16_d  SampleTime=sim_config.Tsample
  To Workspace_I_VSC16_q : ToWorkspace  VariableName=I_VSC16_q  SampleTime=sim_config.Tsample
  To Workspace_I_VSC17_d : ToWorkspace  VariableName=I_VSC17_d  SampleTime=sim_config.Tsample
  To Workspace_I_VSC17_q : ToWorkspace  VariableName=I_VSC17_q  SampleTime=sim_config.Tsample
  To Workspace_I_VSC18_d : ToWorkspace  VariableName=I_VSC18_d  SampleTime=sim_config.Tsample
  To Workspace_I_VSC18_q : ToWorkspace  VariableName=I_VSC18_q  SampleTime=sim_config.Tsample
  To Workspace_I_VSC19_d : ToWorkspace  VariableName=I_VSC19_d  SampleTime=sim_config.Tsample
  To Workspace_I_VSC19_q : ToWorkspace  VariableName=I_VSC19_q  SampleTime=sim_config.Tsample
  To Workspace_I_VSC1_d : ToWorkspace  VariableName=I_VSC1_d  SampleTime=sim_config.Tsample
  To Workspace_I_VSC1_q : ToWorkspace  VariableName=I_VSC1_q  SampleTime=sim_config.Tsample
  To Workspace_I_VSC20_d : ToWorkspace  VariableName=I_VSC20_d  SampleTime=sim_config.Tsample
  To Workspace_I_VSC20_q : ToWorkspace  VariableName=I_VSC20_q  SampleTime=sim_config.Tsample
  To Workspace_I_VSC2_d : ToWorkspace  VariableName=I_VSC2_d  SampleTime=sim_config.Tsample
  To Workspace_I_VSC2_q : ToWorkspace  VariableName=I_VSC2_q  SampleTime=sim_config.Tsample
  To Workspace_I_VSC3_d : ToWorkspace  VariableName=I_VSC3_d  SampleTime=sim_config.Tsample
  To Workspace_I_VSC3_q : ToWorkspace  VariableName=I_VSC3_q  SampleTime=sim_config.Tsample
  To Workspace_I_VSC4_d : ToWorkspace  VariableName=I_VSC4_d  SampleTime=sim_config.Tsample
  To Workspace_I_VSC4_q : ToWorkspace  VariableName=I_VSC4_q  SampleTime=sim_config.Tsample
  To Workspace_I_VSC5_d : ToWorkspace  VariableName=I_VSC5_d  SampleTime=sim_config.Tsample
  To Workspace_I_VSC5_q : ToWorkspace  VariableName=I_VSC5_q  SampleTime=sim_config.Tsample
  To Workspace_I_VSC6_d : ToWorkspace  VariableName=I_VSC6_d  SampleTime=sim_config.Tsample
  To Workspace_I_VSC6_q : ToWorkspace  VariableName=I_VSC6_q  SampleTime=sim_config.Tsample
  To Workspace_I_VSC7_d : ToWorkspace  VariableName=I_VSC7_d  SampleTime=sim_config.Tsample
  To Workspace_I_VSC7_q : ToWorkspace  VariableName=I_VSC7_q  SampleTime=sim_config.Tsample
  To Workspace_I_VSC8_d : ToWorkspace  VariableName=I_VSC8_d  SampleTime=sim_config.Tsample
  To Workspace_I_VSC8_q : ToWorkspace  VariableName=I_VSC8_q  SampleTime=sim_config.Tsample
  To Workspace_I_VSC9_d : ToWorkspace  VariableName=I_VSC9_d  SampleTime=sim_config.Tsample
  To Workspace_I_VSC9_q : ToWorkspace  VariableName=I_VSC9_q  SampleTime=sim_config.Tsample
  To Workspace_NET.vn100d : ToWorkspace  VariableName=vn100d  SampleTime=sim_config.Tsample
  To Workspace_NET.vn100q : ToWorkspace  VariableName=vn100q  SampleTime=sim_config.Tsample
  To Workspace_NET.vn101d : ToWorkspace  VariableName=vn101d  SampleTime=sim_config.Tsample
  To Workspace_NET.vn101q : ToWorkspace  VariableName=vn101q  SampleTime=sim_config.Tsample
